simulink library "ebs_rebuild_generic_std"  (R2016a)
settings: Solver=VariableStepAuto  StartTime=0.0  StopTime=10.0  RelTol=1e-3
undefined symbols (not defined in the file): sMP
(part 2 of 2)

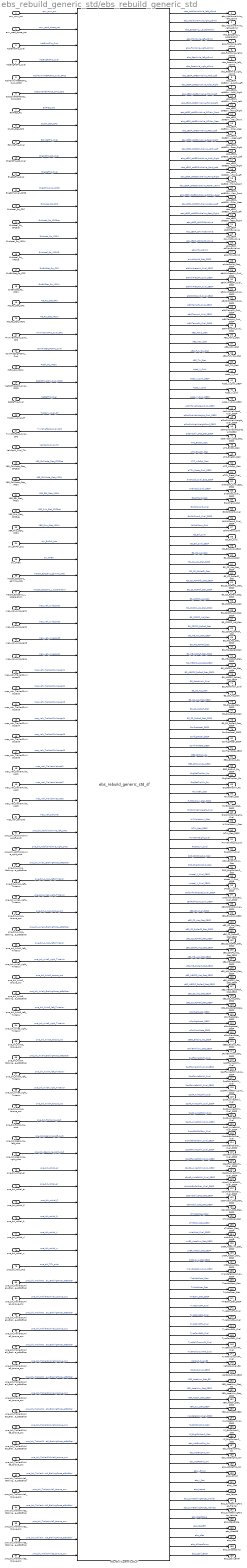
== system ebs_rebuild_generic_std/ebs_rebuild_generic_std ==
  env_curv_pm : Inport
  env_road_slope_pct : Inport  Port=2
  ActlEmotTrq_Cval : Inport  Port=3
  ActlEngPctTrq_Cval : Inport  Port=4
  ActlMaxAvlRetPctTrq_Cval_CPC3 : Inport  Port=5
  aSbspVehBrkForce_Cmd_SDS : Inport  Port=6
  BrkPress_Rq : Inport  Port=7
  Clutch_Stat_CPC : Inport  Port=8
  EdrvRefTrq_Cval : Inport  Port=9
  EngPctTrqActl_Cval : Inport  Port=10
  EngRefTrq_Cval : Inport  Port=11
  EngRPM_Cval_CPC3 : Inport  Port=12
  ExtAccel_Rq_CPC : Inport  Port=13
  ExtAccel_Rq_CPC5ce : Inport  Port=14
  ExtAccel_Rq_VRDU : Inport  Port=15
  ExtAccel_Rq_VRDU3 : Inport  Port=16
  ExtBrkStat_Rq_CPC : Inport  Port=17
  ExtBrkStat_Rq_VRDU : Inport  Port=18
  HB_Rq_Stat_CPC : Inport  Port=19
  HB_Rq_Stat_VRDU : Inport  Port=20
  MinAvlEmotTrq_Cval_CPC : Inport  Port=21
  NomFrictEngPctTrq_Cval : Inport  Port=22
  PkBrk_Rq_VRDU : Inport  Port=23
  RetPctTrqActl2_Cval_CPC3 : Inport  Port=24
  RetRefTrq_Cval : Inport  Port=25
  TrqConv_Cval_PT : Inport  Port=26
  TxInShaftSpd_Cval_CPC : Inport  Port=27
  VehSpd1_Cval_Trlr : Inport  Port=28
  XBR_CtrlMode_Stat_CPC5ce : Inport  Port=29
  XBR_CtrlMode_Stat_VRDU : Inport  Port=30
  XBR_EBI_Stat_VRDU : Inport  Port=31
  XBR_Prio_Stat_CPC5ce : Inport  Port=32
  XBR_Prio_Stat_VRDU : Inport  Port=33
  drv_BrkPdl_pos : Inport  Port=34
  drv_PkBrk : Inport  Port=35
  mec3d_ESCsens_gamma_rate : Inport  Port=36
  mec3d_ESCsens_y_acceleration : Inport  Port=37
  mec_veh_AxleLoad1 : Inport  Port=38
  mec_veh_AxleLoad2 : Inport  Port=39
  mec_veh_AxleLoad3 : Inport  Port=40
  mec_veh_AxleLoad4 : Inport  Port=41
  mec_veh_Trailer02AxleLoad1 : Inport  Port=42
  mec_veh_Trailer02AxleLoad2 : Inport  Port=43
  mec_veh_Trailer02AxleLoad3 : Inport  Port=44
  mec_veh_Trailer02AxleLoad4 : Inport  Port=45
  mec_veh_Trailer02AxleLoad5 : Inport  Port=46
  mec_veh_Trailer02AxleLoad6 : Inport  Port=47
  mec_veh_TrailerAxleLoad1 : Inport  Port=48
  mec_veh_TrailerAxleLoad2 : Inport  Port=49
  mec_veh_TrailerAxleLoad3 : Inport  Port=50
  mec_veh_transVel : Inport  Port=51
  pne_brk_AdditionalAxle_left_pAct : Inport  Port=52
  pne_brk_AdditionalAxle_right_pAct : Inport  Port=53
  pne_brk_Axle1_BrakingForce_at8p5bar : Inport  Port=54
  pne_brk_Axle1_left_Tinterior : Inport  Port=55
  pne_brk_Axle1_right_Tinterior : Inport  Port=56
  pne_brk_Axle1_torque_sns : Inport  Port=57
  pne_brk_Axle2_BrakingForce_at8p5bar : Inport  Port=58
  pne_brk_Axle2_left_Tinterior : Inport  Port=59
  pne_brk_Axle2_right_Tinterior : Inport  Port=60
  pne_brk_Axle2_torque_sns : Inport  Port=61
  pne_brk_Axle3_BrakingForce_at8p5bar : Inport  Port=62
  pne_brk_Axle3_left_Tinterior : Inport  Port=63
  pne_brk_Axle3_right_Tinterior : Inport  Port=64
  pne_brk_Axle3_torque_sns : Inport  Port=65
  pne_brk_Axle4_BrakingForce_at8p5bar : Inport  Port=66
  pne_brk_Axle4_left_Tinterior : Inport  Port=67
  pne_brk_Axle4_right_Tinterior : Inport  Port=68
  pne_brk_Axle4_torque_sns : Inport  Port=69
  pne_brk_FrontAxle_pAct : Inport  Port=70
  pne_brk_RearAxle_left_pAct : Inport  Port=71
  pne_brk_RearAxle_right_pAct : Inport  Port=72
  pne_brk_rotVel_al : Inport  Port=73
  pne_brk_rotVel_ar : Inport  Port=74
  pne_brk_rotVel_fl : Inport  Port=75
  pne_brk_rotVel_fr : Inport  Port=76
  pne_brk_rotVel_rl : Inport  Port=77
  pne_brk_rotVel_rr : Inport  Port=78
  pne_brk_TCV_pAct : Inport  Port=79
  pne_brk_Trailer02Axle1_BrakingForce_at8p5bar : Inport  Port=80
  pne_brk_Trailer02Axle1_torque_sns : Inport  Port=81
  pne_brk_Trailer02Axle2_BrakingForce_at8p5bar : Inport  Port=82
  pne_brk_Trailer02Axle2_torque_sns : Inport  Port=83
  pne_brk_Trailer02Axle3_BrakingForce_at8p5bar : Inport  Port=84
  pne_brk_Trailer02Axle3_torque_sns : Inport  Port=85
  pne_brk_Trailer02Axle4_BrakingForce_at8p5bar : Inport  Port=86
  pne_brk_Trailer02Axle4_torque_sns : Inport  Port=87
  pne_brk_Trailer02Axle5_BrakingForce_at8p5bar : Inport  Port=88
  pne_brk_Trailer02Axle5_torque_sns : Inport  Port=89
  pne_brk_Trailer02Axle6_BrakingForce_at8p5bar : Inport  Port=90
  pne_brk_Trailer02Axle6_torque_sns : Inport  Port=91
  pne_brk_TrailerAxle1_BrakingForce_at8p5bar : Inport  Port=92
  pne_brk_TrailerAxle1_torque_sns : Inport  Port=93
  pne_brk_TrailerAxle2_BrakingForce_at8p5bar : Inport  Port=94
  pne_brk_TrailerAxle2_torque_sns : Inport  Port=95
  pne_brk_TrailerAxle3_BrakingForce_at8p5bar : Inport  Port=96
  pne_brk_TrailerAxle3_torque_sns : Inport  Port=97
  ebs_rebuild_generic_std_sf : S-Function  FunctionName=ebs_rebuild_generic_std_sf  Parameters=s1 s2 p1 p2 p3 p4 p5 p6 p7 p8 p9 p10 p11 p12 p13 p14 p15 p16 p17 p18 p19 p20 p21 p22 p23 p24 p25 p26 p27 p28 p29 p30 p31 p32 p33 p34 p35 p36 p37 p38 p39 p40 p41 p42 p43 p44 p45 p46 p47 p48 p49 p50 p51 p52 p53 p54 p55 p56 p57 p58 p59 p60 p61 p62 p63 p64 p65 p66 p67 p68 p69 p70 p71 p72 p73 p74 p75 p76 p77 p78 p79 p80 p81 p82 p83 p84 p85 p86 p87 p88 p89 p90 p91 p92 p93 p94 p95 p96 p97 p98 p99 p100 p101 p102 p103 p104 p105 p106 p107 p108 p109 p110 p111 p112 p113 p114 p115 p116 p117 p118 p119 p120 p121 p122 p123 p124 p125 p126 p127 p128 p129 p130 p131 p132 p133 p134 p135 p136 p137 p138 p139 p140 p141 p142 p143 p144 p145 p146 p147 p148 p149 p150 p151 p152 p153 p154 p155 p156 p157 p158 p159 p160 p161 p162 p163 p164 p165 p166 p167 p168 p169 p170 p171 p172 p173 p174 p175 p176 p177 p178 p179 p180 p181 p182 p183 p184 p185 p186 p187 p188 p189 p190 p191 p192 p193 p194 p195 p196 p197 p198 p199 p200 p201 p202 p203 p204 p205 p206 p207 p208 p209 p210 p211 p212 p213 p214 p215 p216 p217 p218 p219 p220 p221 p222 p223 p224 p225 p226 p227 p228 p229 p230 p231 p232 p233 p234 p235 p236 p237 p238 p239 p240 p241 p242 p243 p244 p245 p246 p247 p248 p249 p250 p251 p252 p253 p254 p255 p256 p257 p258 p259 p260 p261 p262 p263 p264 p265 p266 p267 p268 p269 p270 p271 p272 p273 p274 p275 p276 p277 p278 p279 p280 p281 p282 p283 p284 p285 p286 p287 p288 p289 p290 p291 p292 p293 p294 p295 p296 p297 p298 p299 p300 p301 p302 p303 p304 p305 p306 p307 p308 p309 p310 p311  SFunctionModules=<binary blob, 502 chars, not shown>  SFunctionDeploymentMode=off  EnableBusSupport=off  mask{s1=s1, s2=s2, initCmd='Parameters_ebs_rebuild_generic_std_sf', p1=p1, p2=p2, p3=p3, p4=p4, p5=p5, p6=p6, p7=p7, p8=p8, p9=p9, p10=p10, p11=p11, p12=p12, p13=p13, p14=p14, p15=p15, p16=p16, p17=p17, p18=p18, p19=p19, p20=p20, p21=p21, p22=p22, p23=p23, p24=p24, p25=p25, p26=p26, p27=p27, p28=p28, p29=p29, p30=p30, p31=p31, p32=p32, p33=p33, p34=p34, p35=p35, p36=p36, p37=p37, p38=p38, p39=p39, p40=p40, p41=p41, p42=p42, p43=p43, p44=p44, p45=p45, p46=p46, p47=p47, p48=p48, p49=p49, p50=p50, p51=p51, p52=p52, p53=p53, p54=p54, p55=p55, p56=p56, p57=p57, p58=p58, p59=p59, p60=p60, p61=p61, p62=p62, p63=p63, p64=p64, p65=p65, p66=p66, p67=p67, p68=p68, p69=p69, p70=p70, p71=p71, p72=p72, p73=p73, p74=p74, p75=p75, p76=p76, p77=p77, p78=p78, p79=p79, p80=p80, p81=p81, p82=p82, p83=p83, p84=p84, p85=p85, p86=p86, p87=p87, p88=p88, p89=p89, p90=p90, p91=p91, p92=p92, p93=p93, p94=p94, p95=p95, p96=p96, p97=p97, p98=p98, p99=p99, p100=p100, p101=p101, p102=p102, p103=p103, p104=p104, p105=p105, p106=p106, p107=p107, p108=p108, p109=p109, p110=p110, p111=p111, p112=p112, p113=p113, p114=p114, p115=p115, p116=p116, p117=p117, p118=p118, p119=p119, p120=p120, p121=p121, p122=p122, p123=p123, p124=p124, p125=p125, p126=p126, p127=p127, p128=p128, p129=p129, p130=p130, p131=p131, p132=p132, p133=p133, p134=p134, p135=p135, p136=p136, p137=p137, p138=p138, p139=p139, p140=p140, p141=p141, p142=p142, p143=p143, p144=p144, p145=p145, p146=p146, p147=p147, p148=p148, p149=p149, p150=p150, p151=p151, p152=p152, p153=p153, p154=p154, p155=p155, p156=p156, p157=p157, p158=p158, p159=p159, p160=p160, p161=p161, p162=p162, p163=p163, p164=p164, p165=p165, p166=p166, p167=p167, p168=p168, p169=p169, p170=p170, p171=p171, p172=p172, p173=p173, p174=p174, p175=p175, p176=p176, p177=p177, p178=p178, p179=p179, p180=p180, p181=p181, p182=p182, p183=p183, p184=p184, p185=p185, p186=p186, p187=p187, p188=p188, p189=p189, p190=p190, p191=p191, p192=p192, p193=p193, p194=p194, p195=p195, p196=p196, p197=p197, p198=p198, p199=p199, p200=p200, p201=p201, p202=p202, p203=p203, p204=p204, p205=p205, p206=p206, p207=p207, p208=p208, p209=p209, p210=p210, p211=p211, p212=p212, p213=p213, p214=p214, p215=p215, p216=p216, p217=p217, p218=p218, p219=p219, p220=p220, p221=p221, p222=p222, p223=p223, p224=p224, p225=p225, p226=p226, p227=p227, p228=p228, p229=p229, p230=p230, p231=p231, p232=p232, p233=p233, p234=p234, p235=p235, p236=p236, p237=p237, p238=p238, p239=p239, p240=p240, p241=p241, p242=p242, p243=p243, p244=p244, p245=p245, p246=p246, p247=p247, p248=p248, p249=p249, p250=p250, p251=p251, p252=p252, p253=p253, p254=p254, p255=p255, p256=p256, p257=p257, p258=p258, p259=p259, p260=p260, p261=p261, p262=p262, p263=p263, p264=p264, p265=p265, p266=p266, p267=p267, p268=p268, p269=p269, p270=p270, p271=p271, p272=p272, p273=p273, p274=p274, p275=p275, p276=p276, p277=p277, p278=p278, p279=p279, p280=p280, p281=p281, p282=p282, p283=p283, p284=p284, p285=p285, p286=p286, p287=p287, p288=p288, p289=p289, p290=p290, p291=p291, p292=p292, p293=p293, p294=p294, p295=p295, p296=p296, p297=p297, p298=p298, p299=p299, p300=p300, p301=p301, p302=p302, p303=p303, p304=p304, p305=p305, p306=p306, p307=p307, p308=p308, p309=p309, p310=p310, p311=p311}
      mask prompts: s1 "Solver Type: settings_iMode [-]"; s2 "Solver Step Size: settings_dt [s]"; initCmd "Initialization command"; p1 "Dimension x-Axis zSoll-Curve [max. 40] export=true name=dim_xAxis_zSoll prio=1 dataSetName=ebs_dummy dataClassType=main dataClassName=main  unit='-' description='Dimension x-Axis zSoll-Curve': BWG.dim_xAxis_zSoll [-]"; p2 "Velocity Offset L1o (km/h) export=true name=ABS_L1o prio=1 dataSetName=veh_dummy dataClassType=veh dataClassName=veh unit='km/h' description='Velocity Offset L1o (km/h)': eBS_veh_Param.ABS_L1o [-]"; p3 "Speed Fraction for Threshold Speed 1 (0.01%) export=true name=ABS_L1v prio=1 dataSetName=veh_dummy dataClassType=veh dataClassName=veh unit='' description='Speed Fraction for Threshold Speed 1 (0.01%)': eBS_veh_Param.ABS_L1v [-]"; p4 "Velocity Offset L2o (km/h) export=true name=ABS_L2o prio=1 dataSetName=veh_dummy dataClassType=veh dataClassName=veh unit='km/h' description='Velocity Offset L2o (km/h)': eBS_veh_Param.ABS_L2o [-]"; p5 "Speed Fraction for Threshold Speed 2 (0.01%) export=true name=ABS_L2v prio=1 dataSetName=veh_dummy dataClassType=veh dataClassName=veh unit='' description='Speed Fraction for Threshold Speed 2 (0.01%)': eBS_veh_Param.ABS_L2v [-]"; p6 "Decceleration Threshold in [g] export=true name=ABS_MinusB prio=1 dataSetName=veh_dummy dataClassType=veh dataClassName=veh unit='' description='Decceleration Threshold in [g]': eBS_veh_Param.ABS_MinusB [-]"; p7 "Acceleration Threshold in [g] export=true name=ABS_PlusB prio=1 dataSetName=veh_dummy dataClassType=veh dataClassName=veh unit='' description='Decceleration Threshold in [g]': eBS_veh_Param.ABS_PlusB [-]"; p8 "Upper Acceleration Threshold in [g] export=true name=ABS_PlusOB prio=1 dataSetName=veh_dummy dataClassType=veh dataClassName=veh unit='' description='Upper Acceleration Threshold in [g]': eBS_veh_Param.ABS_PlusOB [-]"; p9 "Holding Time [ms] export=true name=ABS_THe prio=1 dataSetName=veh_dummy dataClassType=veh dataClassName=veh unit='ms' description='Holding Time [ms]': eBS_veh_Param.ABS_THe [-]"; p10 "Holding Time for Pulsating Pressure Build-Up [ms] export=true name=ABS_TPulHold prio=1 dataSetName=veh_dummy dataClassType=veh dataClassName=veh unit='ms' description='Holding Time for Pulsating Pressure Build-Up [ms]': eBS_veh_Param.ABS_TPulHold [-]"; p11 "Opening Time for Pulsating Pressure Build-Up [ms] export=true name=ABS_TPulOpen prio=1 dataSetName=veh_dummy dataClassType=veh dataClassName=veh unit='ms' description='Opening Time for Pulsating Pressure Build-Up [ms]': eBS_veh_Param.ABS_TPulOpen [-]"; p12 "Minimum Velocity for ABS Activity [km/h] export=true name=ABS_vMin_kmh prio=1 dataSetName=veh_dummy dataClassType=veh dataClassName=veh unit='km/h' description='Minimum Velocity for ABS Activity [km/h]': eBS_veh_Param.ABS_vMin_kmh [-]"; p13 "Trailer ABS Config (0 - none, 1- ABS, 2 - EBS (incl. ABS)), used in pneAux export=true name=flagTrailerABS prio=1 dataSetName=veh_dummy dataClassType=veh dataClassName=veh unit='-' description='Trailer ABS Config (0 - none, 1- ABS, 2 - EBS (incl. ABS))': eBS_veh_Param.flagTrailerABS [-]"; p14 "Dyn. Wheel Radius Front Axle [mm] export=true name=rdynFA prio=1 dataSetName=veh_dummy dataClassType=veh dataClassName=veh unit='mm' description='Dyn. Wheel Radius Front Axle [mm]': eBS_veh_Param.rdynFA [-]"; p15 "Dyn. Wheel Radius Rear Axle [mm] export=true name=rdynRA prio=1 dataSetName=veh_dummy dataClassType=veh dataClassName=veh unit='mm' description='Dyn. Wheel Radius Rear Axle [mm]': eBS_veh_Param.rdynRA [-]"; p16 "Dyn. Wheel Radius Trailer Axle [mm] export=true name=rdynTA prio=1 dataSetName=veh_dummy dataClassType=veh dataClassName=veh unit='mm' description='Dyn. Wheel Radius Trailer Axle [mm]': eBS_veh_Param.rdynTA [-]"; p17 "step Size [s] export=true name=stepSize prio=1 dataSetName=veh_dummy dataClassType=veh dataClassName=veh unit='s' description=' step size [s]': eBS_veh_Param.stepSize [s]"; p18 "ALB Linear Pressure Range p2/p1->1:1 export=true name=ALB_dpMin_bar prio=1 dataSetName=ebs_dummy dataClassType=main dataClassName=main unit=bar description='ALB Linear Pressure Range p2/p1->1:1': eBSParam.ALB_dpMin_bar [-]"; p19 "ALB Maximal Rear Axle Load for p2Max [kg] export=true name=ALB_mRA_Max_kg prio=1 dataSetName=ebs_dummy dataClassType=main dataClassName=main unit=kg description='ALB Maximal Rear Axle Load for p2Max [kg]': eBSParam.ALB_mRA_Max_kg [-]"; p20 "ALB Minimal Rear Axle Load for p2Min [kg] export=true name=ALB_mRA_Min_kg prio=1 dataSetName=ebs_dummy dataClassType=main dataClassName=main unit=kg description='ALB Minimal Rear Axle Load for p2Min [kg]': eBSParam.ALB_mRA_Min_kg [-]"; p21 "ALB Reference Inlet Pressure p1 [bar] export=true name=ALB_p1Ref_bar prio=1 dataSetName=ebs_dummy dataClassType=main dataClassName=main unit=bar description='ALB Reference Inlet Pressure p1 [bar]': eBSParam.ALB_p1Ref_bar [-]"; p22 "ALB Maximum Pressure at mRA_Max_kg [bar] export=true name=ALB_p2Max_bar prio=1 dataSetName=ebs_dummy dataClassType=main dataClassName=main unit=bar description='ALB Maximum Pressure at mRA_Max_kg [bar]': eBSParam.ALB_p2Max_bar [-]"; p23 "ALB Minimum Pressure at mRA_Min [bar] export=true name=ALB_p2Min_bar prio=1 dataSetName=ebs_dummy dataClassType=main dataClassName=main unit=bar description='ALB Minimum Pressure at mRA_Min [bar]': eBSParam.ALB_p2Min_bar [-]"; p24 "Maximum Friction Coefficient Rear Axle export=true name=EBI_mueMax prio=1 dataSetName=ebs_dummy dataClassType=main dataClassName=main unit='-' description='Maximum Friction Coefficient Rear Axle': eBSParam.EBI_mueMax [-]"; p25 "Minum Initial Velocity [km/h] (eBIActive>EBI_vMin_kmh) export=true name=EBI_vMin_kmh prio=1 dataSetName=ebs_dummy dataClassType=main dataClassName=main unit='km/h' description='Minum Initial Velocity [km/h] (eBIActive>EBI_vMin_kmh)': eBSParam.EBI_vMin_kmh [-]"; p26 "Vehicle with ABS-Brake System [0-false,1-true] export=true name=flag_ABS prio=1 dataSetName=ebs_dummy dataClassType=main dataClassName=main unit='-' description='Vehicle with ABS-Brake System [0-false,1-true]': eBSParam.flag_ABS [-]"; p27 "Flag Downhill Drive Test [0-false,1-true] export=true name=flag_DownhillDriveTest prio=1 dataSetName=ebs_dummy dataClassType=main dataClassName=main unit='-' description='Flag Downhill Drive Test [0-false,1-true]': eBSParam.flag_DownhillDriveTest [-]"; p28 "Endurance Brake Integration (EBI) [0-no EBI,1-EBI, base deceleration of 2% by service brake, 2- EBI 100%, 3 - prior endurance brake activation, 4 - EBI Bus mode] export=true name=flag_EBI prio=1 dataSetName=ebs_dummy dataClassType=main dataClassName=main unit='-' description='Endurance Brake Integration (EBI) [0-no EBI,1-EBI, base deceleration of 2% by service brake, 2- EBI 100%, 3 - prior endurance brake activation, 4 - EBI Bus mode]': eBSParam.flag_EBI [-]"; p29 "Slope Compensation Active [0 - false,1 - true] export=true name=flag_SlopeCompActive prio=1 dataSetName=ebs_dummy dataClassType=main dataClassName=main unit='-' description='Slope Compensation Active [0 - false,1 - true]': eBSParam.flag_SlopeCompActive [-]"; p30 "Transmission Ratio EMot - Axle [-] export=true name=mec_iDiffAxle prio=1 dataSetName=ebs_dummy dataClassType=main dataClassName=main unit='' description='Transmission Ratio EMot - Axle [-]': eBSParam.mec_iDiffAxle [-]"; p31 "Recuperation value for full brake pedal actuation [Nm] export=true name=Recuperation_end prio=1 dataSetName=ebs_dummy dataClassType=main dataClassName=main unit=kg description='Recuperation value for inital brake pedal actuation [Nm] ': eBSParam.Recuperation_end [-]"; p32 "Recuperation value for inital brake pedal actuation [Nm] export=true name=Recuperation_initial prio=1 dataSetName=ebs_dummy dataClassType=main dataClassName=main unit=kg description='Recuperation value for inital brake pedal actuation [Nm] ': eBSParam.Recuperation_initial [-]"; p33 "aAutoOpMd_Stat_SBSP export=true name=aAutoOpMd_Stat_SBSP prio=1 dataSetName=std dataClassType=initIO dataClassName=initIO unit='-' description='aAutoOpMd_Stat_SBSP': IO_EBS_InputSignals.aAutoOpMd_Stat_SBSP_0 [-]"; p34 "aBrkAirPressAA_Cval_SBSP export=true name=aBrkAirPressAA_Cval_SBSP prio=1 dataSetName=std dataClassType=initIO dataClassName=initIO unit='kPa' description='aBrkAirPressAA_Cval_SBSP': IO_EBS_InputSignals.aBrkAirPressAA_Cval_SBSP_0 [-]"; p35 "aBrkAirPressFA_Cval_SBSP export=true name=aBrkAirPressFA_Cval_SBSP prio=1 dataSetName=std dataClassType=initIO dataClassName=initIO unit='kPa' description='aBrkAirPressFA_Cval_SBSP': IO_EBS_InputSignals.aBrkAirPressFA_Cval_SBSP_0 [-]"; p36 "aBrkAirPressRA_Cval_SBSP export=true name=aBrkAirPressRA_Cval_SBSP prio=1 dataSetName=std dataClassType=initIO dataClassName=initIO unit='kPa' description='aBrkAirPressRA_Cval_SBSP': IO_EBS_InputSignals.aBrkAirPressRA_Cval_SBSP_0 [-]"; p37 "aBrkPdlPosn3_Cval_SBSP export=true name=aBrkPdlPosn3_Cval_SBSP prio=1 dataSetName=std dataClassType=initIO dataClassName=initIO unit='%' description='aBrkPdlPosn3_Cval_SBSP': IO_EBS_InputSignals.aBrkPdlPosn3_Cval_SBSP_0 [-]"; p38 "aBrkTempFA_Cval_SBSP export=true name=aBrkTempFA_Cval_SBSP prio=1 dataSetName=std dataClassType=initIO dataClassName=initIO unit='degC' description='aBrkTempFA_Cval_SBSP': IO_EBS_InputSignals.aBrkTempFA_Cval_SBSP_0 [-]"; p39 "aBrkTempIA_Cval_SBSP export=true name=aBrkTempIA_Cval_SBSP prio=1 dataSetName=std dataClassType=initIO dataClassName=initIO unit='degC' description='aBrkTempIA_Cval_SBSP': IO_EBS_InputSignals.aBrkTempIA_Cval_SBSP_0 [-]"; p40 "aBrkTempRA_Cval_SBSP export=true name=aBrkTempRA_Cval_SBSP prio=1 dataSetName=std dataClassType=initIO dataClassName=initIO unit='degC' description='aBrkTempRA_Cval_SBSP': IO_EBS_InputSignals.aBrkTempRA_Cval_SBSP_0 [-]"; p41 "ABS_Actv2_Stat export=true name=ABS_Actv2_Stat prio=1 dataSetName=std dataClassType=initIO dataClassName=initIO unit='-' description='ABS_Actv2_Stat': IO_EBS_InputSignals.ABS_Actv2_Stat_0 [-]"; p42 "ABS_Actv_Stat export=true name=ABS_Actv_Stat prio=1 dataSetName=std dataClassType=initIO dataClassName=initIO unit='-' description='ABS_Actv_Stat': IO_EBS_InputSignals.ABS_Actv_Stat_0 [-]"; p43 "ABS_FullyOp_Stat export=true name=ABS_FullyOp_Stat prio=1 dataSetName=std dataClassType=initIO dataClassName=initIO unit='-' description='ABS_FullyOp_Stat': IO_EBS_InputSignals.ABS_FullyOp_Stat_0 [-]"; p44 "ABS_Trlr_Stat export=true name=ABS_Trlr_Stat prio=1 dataSetName=std dataClassType=initIO dataClassName=initIO unit='-' description='ABS_Trlr_Stat': IO_EBS_InputSignals.ABS_Trlr_Stat_0 [-]"; p45 "ABS61449S_E_LongitudAcc, 255 SNA; export=true name=Accel_X_Cval prio=1 dataSetName=std dataClassType=initIO dataClassName=initIO unit='m/s^2' description='ABS61449S_E_LongitudAcc, 255 SNA;': IO_EBS_InputSignals.Accel_X_Cval_0 [-]"; p46 "ABS61449S_E_LongitudAcc, 255 SNA; export=true name=Accel_X_Cval_SBSP prio=1 dataSetName=std dataClassType=initIO dataClassName=initIO unit='m/s^2' description='ABS61449S_E_LongitudAcc, 255 SNA;': IO_EBS_InputSignals.Accel_X_Cval_SBSP_0 [-]"; p47 "Accel_Y_Cval export=true name=Accel_Y_Cval prio=1 dataSetName=std dataClassType=initIO dataClassName=initIO unit=m/s^2 description='Accel_Y_Cval': IO_EBS_InputSignals.Accel_Y_Cval_0 [-]"; p48 "Accel_Y_Cval_SBSP export=true name=Accel_Y_Cval_SBSP prio=1 dataSetName=std dataClassType=initIO dataClassName=initIO unit=m/s^2 description='Accel_Y_Cval_SBSP': IO_EBS_InputSignals.Accel_Y_Cval_SBSP_0 [-]"; p49 "ActlEmotTrq_Cval (init) export=true name=ActlEmotTrq_Cval prio=1 dataSetName=std dataClassType=initIO dataClassName=initIO unit='-' description='ActlEmotTrq_Cval (init)': IO_EBS_InputSignals.ActlEmotTrq_Cval_0 [-]"; p50 "ActlEngPctTrq_Cval export=true name=ActlEngPctTrq_Cval prio=1 dataSetName=std dataClassType=initIO dataClassName=initIO unit='-' description='ActlEngPctTrq_Cval': IO_EBS_InputSignals.ActlEngPctTrq_Cval_0 [-]"; p51 "ActlMaxAvlRetPctTrq_Cval_CPC3 export=true name=ActlMaxAvlRetPctTrq_Cval_CPC3 prio=1 dataSetName=std dataClassType=initIO dataClassName=initIO unit='-' description='ActlMaxAvlRetPctTrq_Cval_CPC3': IO_EBS_InputSignals.ActlMaxAvlRetPctTrq_Cval_CPC3_0 [-]"; p52 "AddInfoVehSped_Cval_SBSP (init) export=true name=AddInfoVehSped_Cval_SBSP prio=1 dataSetName=std dataClassType=initIO dataClassName=initIO unit='' description='AddInfoVehSped_Cval_SBSP': IO_EBS_InputSignals.AddInfoVehSped_Cval_SBSP_0 [-]"; p53 "aGroCmbVehWeight_Cval_SBSP export=true name=aGroCmbVehWeight_Cval_SBSP prio=1 dataSetName=std dataClassType=initIO dataClassName=initIO unit='kg' description='aGroCmbVehWeight_Cval_SBSP': IO_EBS_InputSignals.aGroCmbVehWeight_Cval_SBSP_0 [-]"; p54 "aGroCmbVehWeightConf_SBSP export=true name=aGroCmbVehWeightConf_SBSP prio=1 dataSetName=std dataClassType=initIO dataClassName=initIO unit='%' description='Vehicle Mass estimate confidence factor': IO_EBS_InputSignals.aGroCmbVehWeightConf_SBSP_0 [-]"; p55 "aSbspVehBrkForce_Cmd_SDS export=true name=aSbspVehBrkForce_Cmd_SDS prio=1 dataSetName=std dataClassType=initIO dataClassName=initIO unit='N' description='aSbspVehBrkForce_Cmd_SDS': IO_EBS_InputSignals.aSbspVehBrkForce_Cmd_SDS_0 [-]"; p56 "aStandstill_Dtct_Stat_SBSP export=true name=aStandstill_Dtct_Stat_SBSP prio=1 dataSetName=std dataClassType=initIO dataClassName=initIO unit='-' description='Standstill detected Current state': IO_EBS_InputSignals.aStandstill_Dtct_Stat_SBSP_0 [-]"; p57 "ATC_BrkCtrl_Stat export=true name=ATC_BrkCtrl_Stat prio=1 dataSetName=std dataClassType=initIO dataClassName=initIO unit='-' description='ATC_BrkCtrl_Stat': IO_EBS_InputSignals.ATC_BrkCtrl_Stat_0 [-]"; p58 "ATC_EngCtrl_Stat export=true name=ATC_EngCtrl_Stat prio=1 dataSetName=std dataClassType=initIO dataClassName=initIO unit='-' description='ATC_EngCtrl_Stat': IO_EBS_InputSignals.ATC_EngCtrl_Stat_0 [-]"; p59 "ATC_InfoSgl_Stat export=true name=ATC_InfoSgl_Stat prio=1 dataSetName=std dataClassType=initIO dataClassName=initIO unit='-' description='ATC_InfoSgl_Stat': IO_EBS_InputSignals.ATC_InfoSgl_Stat_0 [-]"; p60 "aTCV_Press_Cval_SBSP export=true name=aTCV_Press_Cval_SBSP prio=1 dataSetName=std dataClassType=initIO dataClassName=initIO unit='kPa' description='aTCV_Press_Cval_SBSP': IO_EBS_InputSignals.aTCV_Press_Cval_SBSP_0 [-]"; p61 "aVehSpd_Cval_E2E_SBSP export=true name=aVehSpd_Cval_E2E_SBSP prio=1 dataSetName=std dataClassType=initIO dataClassName=initIO unit='km/h' description='aVehSpd_Cval_E2E_SBSP': IO_EBS_InputSignals.aVehSpd_Cval_E2E_SBSP_0 [-]"; p62 "aVehSpd_Cval_SBSP export=true name=aVehSpd_Cval_SBSP prio=1 dataSetName=std dataClassType=initIO dataClassName=initIO unit='km/h' description='Vehicle Speed Current value': IO_EBS_InputSignals.aVehSpd_Cval_SBSP_0 [-]"; p63 "BlockTend_Stat export=true name=BlockTend_Stat prio=1 dataSetName=std dataClassType=initIO dataClassName=initIO unit='-' description='BlockTend_Stat': IO_EBS_InputSignals.BlockTend_Stat_0 [-]"; p64 "Brake Pedal Position 3 Current value (an CPC3) export=true name=BrkPdlPosn3_Cval prio=1 dataSetName=std dataClassType=initIO dataClassName=initIO unit='%' description='Brake Pedal Position 3 Current value (an CPC3)': IO_EBS_InputSignals.BrkPdlPosn3_Cval_0 [-]"; p65 "Brake Pedal Position 3 Current value (an CPC3) export=true name=BrkPdlPosn3_Cval_SBSP prio=1 dataSetName=std dataClassType=initIO dataClassName=initIO unit='%' description='Brake Pedal Position 3 Current value (an CPC3) SBSP': IO_EBS_InputSignals.BrkPdlPosn3_Cval_SBSP_0 [-]"; p66 "Brake Pedal Position Current value (an CGW) export=true name=BrkPdlPosn_Cval prio=1 dataSetName=std dataClassType=initIO dataClassName=initIO unit='%' description='Brake Pedal Position Current value (an CGW)': IO_EBS_InputSignals.BrkPdlPosn_Cval_0 [-]"; p67 "BrkPress_Rq export=true name=BrkPress_Rq prio=1 dataSetName=std dataClassType=initIO dataClassName=initIO unit='-' description='BrkPress_Rq': IO_EBS_InputSignals.BrkPress_Rq_0 [-]"; p68 "Brake Current value, 254 ERR; 255 SNA; export=true name=BS_Brk_Cval prio=1 dataSetName=std dataClassType=initIO dataClassName=initIO unit='%' description='Brake Current value, 254 ERR; 255 SNA;': IO_EBS_InputSignals.BS_Brk_Cval_0 [-]"; p69 "Brake Current value, 254 ERR; 255 SNA; export=true name=BS_Brk_Cval_SBSP prio=1 dataSetName=std dataClassType=initIO dataClassName=initIO unit='%' description='Brake Current value, 254 ERR; 255 SNA; SBSP': IO_EBS_InputSignals.BS_Brk_Cval_SBSP_0 [-]"; p70 "BS_CS_Acc_Stat export=true name=BS_CS_Acc_Stat prio=1 dataSetName=std dataClassType=initIO dataClassName=initIO unit='-' description='BS_CSCPC_Acc_Stat': IO_EBS_InputSignals.BS_CS_Acc_Stat_0 [-]"; p71 "BS_CS_Acc_Stat_SBSP export=true name=BS_CS_Acc_Stat_SBSP prio=1 dataSetName=std dataClassType=initIO dataClassName=initIO unit='-' description='BS_CSCPC_Acc_Stat': IO_EBS_InputSignals.BS_CS_Acc_Stat_SBSP_0 [-]"; p72 "BS_CS_RqPerf2_Stat export=true name=BS_CS_RqPerf2_Stat prio=1 dataSetName=std dataClassType=initIO dataClassName=initIO unit='-' description='BS_CS_RqPerf2_Stat': IO_EBS_InputSignals.BS_CS_RqPerf2_Stat_0 [-]"; p73 "BS_CS_RqPerf2_Stat_SBSP export=true name=BS_CS_RqPerf2_Stat_SBSP prio=1 dataSetName=std dataClassType=initIO dataClassName=initIO unit='-' description='BS_CS_RqPerf2_Stat_SBSP': IO_EBS_InputSignals.BS_CS_RqPerf2_Stat_SBSP_0 [-]"; p74 "BS_CS_RqPerf_Stat_SBSP export=true name=BS_CS_RqPerf_Stat_SBSP prio=1 dataSetName=std dataClassType=initIO dataClassName=initIO unit='-' description='BS_CS_RqPerf_Stat_SBSP': IO_EBS_InputSignals.BS_CS_RqPerf_Stat_SBSP_0 [-]"; p75 "BS_CSCPC_Acc_Stat export=true name=BS_CSCPC_Acc_Stat prio=1 dataSetName=std dataClassType=initIO dataClassName=initIO unit='-' description='BS_CSCPC_Acc_Stat': IO_EBS_InputSignals.BS_CSCPC_Acc_Stat_0 [-]"; p76 "BS_CSCPC_Acc_Stat_SBSP export=true name=BS_CSCPC_Acc_Stat_SBSP prio=1 dataSetName=std dataClassType=initIO dataClassName=initIO unit='-' description='BS_CSCPC_Acc_Stat_SBSP': IO_EBS_InputSignals.BS_CSCPC_Acc_Stat_SBSP_0 [-]"; p77 "BS_CSCPC_Intf_Stat export=true name=BS_CSCPC_Intf_Stat prio=1 dataSetName=std dataClassType=initIO dataClassName=initIO unit='-' description='BS_CSCPC_Intf_Stat': IO_EBS_InputSignals.BS_CSCPC_Intf_Stat_0 [-]"; p78 "BS_CSCPC_RqPerf_Stat export=true name=BS_CSCPC_RqPerf_Stat prio=1 dataSetName=std dataClassType=initIO dataClassName=initIO unit='-' description='BS_CSCPC_RqPerf_Stat': IO_EBS_InputSignals.BS_CSCPC_RqPerf_Stat_0 [-]"; p79 "BS_HB_Acc_Stat_SBSP export=true name=BS_HB_Acc_Stat_SBSP prio=1 dataSetName=std dataClassType=initIO dataClassName=initIO unit='-' description='BS_HB_Acc_Stat_SBSP': IO_EBS_InputSignals.BS_HB_Acc_Stat_SBSP_0 [-]"; p80 "Brake Current value, 254 ERR; 255 SNA; export=true name=BS_HB_RqPerf_Stat prio=1 dataSetName=std dataClassType=initIO dataClassName=initIO unit='-' description='Brake Current value, 254 ERR; 255 SNA;': IO_EBS_InputSignals.BS_HB_RqPerf_Stat_0 [-]"; p81 "Brake Current value, 254 ERR; 255 SNA; export=true name=BS_HB_RqPerf_Stat_SBSP prio=1 dataSetName=std dataClassType=initIO dataClassName=initIO unit='-' description='Brake Current value, 254 ERR; 255 SNA; SBSP': IO_EBS_InputSignals.BS_HB_RqPerf_Stat_SBSP_0 [-]"; p82 "BS_HBCPC_Acc_Stat_SBSP export=true name=BS_HBCPC_Acc_Stat_SBSP prio=1 dataSetName=std dataClassType=initIO dataClassName=initIO unit='-' description='BS_HBCPC_Acc_Stat_SBSP': IO_EBS_InputSignals.BS_HBCPC_Acc_Stat_SBSP_0 [-]"; p83 "BS_HBCPC_RqPerf_Stat_SBSP export=true name=BS_HBCPC_RqPerf_Stat_SBSP prio=1 dataSetName=std dataClassType=initIO dataClassName=initIO unit='-' description='BS_HBCPC_RqPerf_Stat_SBSP': IO_EBS_InputSignals.BS_HBCPC_RqPerf_Stat_SBSP_0 [-]"; p84 "Road inclination current value (calculated), 254 ERR; 255 SNA; export=true name=BS_RoadIncln_Cval prio=1 dataSetName=std dataClassType=initIO dataClassName=initIO unit='%' description='Road inclination current value (calculated), 254 ERR; 255 SNA;': IO_EBS_InputSignals.BS_RoadIncln_Cval_0 [-]"; p85 "BS_SS_Acc_Stat export=true name=BS_SS_Acc_Stat prio=1 dataSetName=std dataClassType=initIO dataClassName=initIO unit='-' description='BS_CSCPC_Acc_Stat': IO_EBS_InputSignals.BS_SS_Acc_Stat_0 [-]"; p86 "BS_SS_Acc_Stat_SBSP export=true name=BS_SS_Acc_Stat_SBSP prio=1 dataSetName=std dataClassType=initIO dataClassName=initIO unit='-' description='BS_CSCPC_Acc_Stat': IO_EBS_InputSignals.BS_SS_Acc_Stat_SBSP_0 [-]"; p87 "BS_SS_RqPerf_Stat export=true name=BS_SS_RqPerf_Stat prio=1 dataSetName=std dataClassType=initIO dataClassName=initIO unit='-' description='BS_SS_RqPerf_Stat': IO_EBS_InputSignals.BS_SS_RqPerf_Stat_0 [-]"; p88 "BS_SS_RqPerf_Stat_SBSP export=true name=BS_SS_RqPerf_Stat_SBSP prio=1 dataSetName=std dataClassType=initIO dataClassName=initIO unit='-' description='BS_SS_RqPerf_Stat_SBSP': IO_EBS_InputSignals.BS_SS_RqPerf_Stat_SBSP_0 [-]"; p89 "Clutch_Stat_CPC (init) export=true name=Clutch_Stat_CPC prio=1 dataSetName=std dataClassType=initIO dataClassName=initIO unit='-' description='Clutch_Stat_CPC (init)': IO_EBS_InputSignals.Clutch_Stat_CPC_0 [-]"; p90 "ConfLatAccel_SBSP (init) export=true name=ConfLatAccel_SBSP prio=1 dataSetName=std dataClassType=initIO dataClassName=initIO unit='%' description='ConfLatAccel_SBSP': IO_EBS_InputSignals.ConfLatAccel_SBSP_0 [-]"; p91 "ConfLgtAccel_SBSP (init) export=true name=ConfLgtAccel_SBSP prio=1 dataSetName=std dataClassType=initIO dataClassName=initIO unit='%' description='ConfLgtAccel_SBSP': IO_EBS_InputSignals.ConfLgtAccel_SBSP_0 [-]"; p92 "ConfYawRate_SBSP (init) export=true name=ConfYawRate_SBSP prio=1 dataSetName=std dataClassType=initIO dataClassName=initIO unit='%' description='ConfYawRate_SBSP': IO_EBS_InputSignals.ConfYawRate_SBSP_0 [-]"; p93 "drv_BrkPdl_pos export=true name=drv_BrkPdl_pos prio=1 dataSetName=std dataClassType=initIO dataClassName=initIO unit='-' description='drv_BrkPdl_pos': IO_EBS_InputSignals.drv_BrkPdl_pos_0 [-]"; p94 "drv_PkBrk export=true name=drv_PkBrk prio=1 dataSetName=std dataClassType=initIO dataClassName=initIO unit='-' description='drv_PkBrk': IO_EBS_InputSignals.drv_PkBrk_0 [-]"; p95 "ebs_ActlEmotTrq_Nm export=true name=ebs_ActlEmotTrq_Nm prio=1 dataSetName=std dataClassType=initIO dataClassName=initIO unit=Nm description='ebs_ActlEmotTrq_Nm': IO_EBS_InputSignals.ebs_ActlEmotTrq_Nm_0 [-]"; p96 "ebs_ActlEngTrq_Nm export=true name=ebs_ActlEngTrq_Nm prio=1 dataSetName=std dataClassType=initIO dataClassName=initIO unit=Nm description='ebs_ActlEngTrq_Nm': IO_EBS_InputSignals.ebs_ActlEngTrq_Nm_0 [-]"; p97 "ebs_ActlRetTrq_Nm export=true name=ebs_ActlRetTrq_Nm prio=1 dataSetName=std dataClassType=initIO dataClassName=initIO unit=Nm description='ebs_ActlRetTrq_Nm': IO_EBS_InputSignals.ebs_ActlRetTrq_Nm_0 [-]"; p98 "ebs_AdditionalAxle_left_pDmd (init) export=true name=ebs_AdditionalAxle_left_pDmd prio=1 dataSetName=std dataClassType=initIO dataClassName=initIO unit='-' description='ebs_AdditionalAxle_left_pDmd': IO_EBS_InputSignals.ebs_AdditionalAxle_left_pDmd_0 [-]"; p99 "ebs_AdditionalAxle_right_pDmd (init) export=true name=ebs_AdditionalAxle_right_pDmd prio=1 dataSetName=std dataClassType=initIO dataClassName=initIO unit='-' description='ebs_AdditionalAxle_right_pDmd': IO_EBS_InputSignals.ebs_AdditionalAxle_right_pDmd_0 [-]"; p100 "EBS Brake Switch 2 Request state for DTR+, 0 NPSD; 1 PSD; 2 ERR; 3 SNA; export=true name=EBS_BrkSw2_Rq prio=1 dataSetName=std dataClassType=initIO dataClassName=initIO unit='-' description='EBS Brake Switch 2 Request state for DTR+, 0 NPSD; 1 PSD; 2 ERR; 3 SNA;': IO_EBS_InputSignals.EBS_BrkSw2_Rq_0 [-]"; p101 "EBS Brake Switch 2 Request state for DTR+, 0 NPSD; 1 PSD; 2 ERR; 3 SNA; export=true name=EBS_BrkSw2_Rq_SBSP prio=1 dataSetName=std dataClassType=initIO dataClassName=initIO unit='-' description='EBS Brake Switch 2 Request state for DTR+, 0 NPSD; 1 PSD; 2 ERR; 3 SNA;': IO_EBS_InputSignals.EBS_BrkSw2_Rq_SBSP_0 [-]"; p102 "ebs_ESCsens_y_acceleration export=true name=ebs_ESCsens_y_acceleration prio=1 dataSetName=std dataClassType=initIO dataClassName=initIO unit='m/s^2' description='ebs_ESCsens_y_acceleration': IO_EBS_InputSignals.ebs_ESCsens_y_acceleration_0 [-]"; p103 "ebs_FrontAxle_left_pDmd (init) export=true name=ebs_FrontAxle_left_pDmd prio=1 dataSetName=std dataClassType=initIO dataClassName=initIO unit='-' description='ebs_FrontAxle_left_pDmd': IO_EBS_InputSignals.ebs_FrontAxle_left_pDmd_0 [-]"; p104 "ebs_FrontAxle_right_pDmd (init) export=true name=ebs_FrontAxle_right_pDmd prio=1 dataSetName=std dataClassType=initIO dataClassName=initIO unit='-' description='ebs_FrontAxle_right_pDmd': IO_EBS_InputSignals.ebs_FrontAxle_right_pDmd_0 [-]"; p105 "ebs_i_Emot export=true name=ebs_i_Emot prio=1 dataSetName=std dataClassType=initIO dataClassName=initIO unit='-' description='ebs_i_Emot': IO_EBS_InputSignals.ebs_i_Emot_0 [-]"; p106 "ebs_i_Ret export=true name=ebs_i_Ret prio=1 dataSetName=std dataClassType=initIO dataClassName=initIO unit='-' description='ebs_i_Ret': IO_EBS_InputSignals.ebs_i_Ret_0 [-]"; p107 "ebs_kappa export=true name=ebs_kappa prio=1 dataSetName=std dataClassType=initIO dataClassName=initIO unit='-' description='ebs_kappa': IO_EBS_InputSignals.ebs_kappa_0 [-]"; p108 "ebs_RearAxle_left_pDmd (init) export=true name=ebs_RearAxle_left_pDmd prio=1 dataSetName=std dataClassType=initIO dataClassName=initIO unit='-' description='ebs_RearAxle_left_pDmd': IO_EBS_InputSignals.ebs_RearAxle_left_pDmd_0 [-]"; p109 "ebs_RearAxle_right_pDmd (init) export=true name=ebs_RearAxle_right_pDmd prio=1 dataSetName=std dataClassType=initIO dataClassName=initIO unit='-' description='ebs_RearAxle_right_pDmd': IO_EBS_InputSignals.ebs_RearAxle_right_pDmd_0 [-]"; p110 "ebs_sBSP_stABSInValve_Addl_Left export=true name=ebs_sBSP_stABSInValve_Addl_Left prio=1 dataSetName=std dataClassType=initIO dataClassName=initIO unit='-' description='ebs_sBSP_stABSInValve_Addl_Left': IO_EBS_InputSignals.ebs_sBSP_stABSInValve_Addl_Left_0 [-]"; p111 "ebs_sBSP_stABSInValve_Addl_Right export=true name=ebs_sBSP_stABSInValve_Addl_Right prio=1 dataSetName=std dataClassType=initIO dataClassName=initIO unit='-' description='ebs_sBSP_stABSInValve_Addl_Right': IO_EBS_InputSignals.ebs_sBSP_stABSInValve_Addl_Right_0 [-]"; p112 "ebs_sBSP_stABSInValve_Front_Left export=true name=ebs_sBSP_stABSInValve_Front_Left prio=1 dataSetName=std dataClassType=initIO dataClassName=initIO unit='-' description='ebs_sBSP_stABSInValve_Front_Left': IO_EBS_InputSignals.ebs_sBSP_stABSInValve_Front_Left_0 [-]"; p113 "ebs_sBSP_stABSInValve_Front_Right export=true name=ebs_sBSP_stABSInValve_Front_Right prio=1 dataSetName=std dataClassType=initIO dataClassName=initIO unit='-' description='ebs_sBSP_stABSInValve_Front_Right': IO_EBS_InputSignals.ebs_sBSP_stABSInValve_Front_Right_0 [-]"; p114 "ebs_sBSP_stABSInValve_RCMax_Front (init),   export=true name=ebs_sBSP_stABSInValve_RCMax_Front prio=1 dataSetName=std dataClassType=initIO dataClassName=initIO unit='-' description=' ': IO_EBS_InputSignals.ebs_sBSP_stABSInValve_RCMax_Front_0 [-]"; p115 "ebs_sBSP_stABSInValve_RCMax_Rear (init),   export=true name=ebs_sBSP_stABSInValve_RCMax_Rear prio=1 dataSetName=std dataClassType=initIO dataClassName=initIO unit='-' description=' ': IO_EBS_InputSignals.ebs_sBSP_stABSInValve_RCMax_Rear_0 [-]"; p116 "ebs_sBSP_stABSInValve_Rear_Left export=true name=ebs_sBSP_stABSInValve_Rear_Left prio=1 dataSetName=std dataClassType=initIO dataClassName=initIO unit='-' description='ebs_sBSP_stABSInValve_Rear_Left': IO_EBS_InputSignals.ebs_sBSP_stABSInValve_Rear_Left_0 [-]"; p117 "ebs_sBSP_stABSInValve_Rear_Right export=true name=ebs_sBSP_stABSInValve_Rear_Right prio=1 dataSetName=std dataClassType=initIO dataClassName=initIO unit='-' description='ebs_sBSP_stABSInValve_Rear_Right': IO_EBS_InputSignals.ebs_sBSP_stABSInValve_Rear_Right_0 [-]"; p118 "ebs_sBSP_stABSOutValve_Addl_Left export=true name=ebs_sBSP_stABSOutValve_Addl_Left prio=1 dataSetName=std dataClassType=initIO dataClassName=initIO unit='-' description='ebs_sBSP_stABSOutValve_Addl_Left': IO_EBS_InputSignals.ebs_sBSP_stABSOutValve_Addl_Left_0 [-]"; p119 "ebs_sBSP_stABSOutValve_Addl_Right export=true name=ebs_sBSP_stABSOutValve_Addl_Right prio=1 dataSetName=std dataClassType=initIO dataClassName=initIO unit='-' description='ebs_sBSP_stABSOutValve_Addl_Right': IO_EBS_InputSignals.ebs_sBSP_stABSOutValve_Addl_Right_0 [-]"; p120 "ebs_sBSP_stABSOutValve_Front_Left export=true name=ebs_sBSP_stABSOutValve_Front_Left prio=1 dataSetName=std dataClassType=initIO dataClassName=initIO unit='-' description='ebs_sBSP_stABSOutValve_Front_Left': IO_EBS_InputSignals.ebs_sBSP_stABSOutValve_Front_Left_0 [-]"; p121 "ebs_sBSP_stABSOutValve_Front_Right export=true name=ebs_sBSP_stABSOutValve_Front_Right prio=1 dataSetName=std dataClassType=initIO dataClassName=initIO unit='-' description='ebs_sBSP_stABSOutValve_Front_Right': IO_EBS_InputSignals.ebs_sBSP_stABSOutValve_Front_Right_0 [-]"; p122 "ebs_sBSP_stABSOutValve_RCMax_Front (init),   export=true name=ebs_sBSP_stABSOutValve_RCMax_Front prio=1 dataSetName=std dataClassType=initIO dataClassName=initIO unit='-' description=' ': IO_EBS_InputSignals.ebs_sBSP_stABSOutValve_RCMax_Front_0 [-]"; p123 "ebs_sBSP_stABSOutValve_RCMax_Rear (init),   export=true name=ebs_sBSP_stABSOutValve_RCMax_Rear prio=1 dataSetName=std dataClassType=initIO dataClassName=initIO unit='-' description=' ': IO_EBS_InputSignals.ebs_sBSP_stABSOutValve_RCMax_Rear_0 [-]"; p124 "ebs_sBSP_stABSOutValve_Rear_Left export=true name=ebs_sBSP_stABSOutValve_Rear_Left prio=1 dataSetName=std dataClassType=initIO dataClassName=initIO unit='-' description='ebs_sBSP_stABSOutValve_Rear_Left': IO_EBS_InputSignals.ebs_sBSP_stABSOutValve_Rear_Left_0 [-]"; p125 "ebs_sBSP_stABSOutValve_Rear_Right export=true name=ebs_sBSP_stABSOutValve_Rear_Right prio=1 dataSetName=std dataClassType=initIO dataClassName=initIO unit='-' description='ebs_sBSP_stABSOutValve_Rear_Right': IO_EBS_InputSignals.ebs_sBSP_stABSOutValve_Rear_Right_0 [-]"; p126 "ebs_sBSP_stAPCVBuValve export=true name=ebs_sBSP_stAPCVBuValve prio=1 dataSetName=std dataClassType=initIO dataClassName=initIO unit='-' description='ebs_sBSP_stAPCVBuValve': IO_EBS_InputSignals.ebs_sBSP_stAPCVBuValve_0 [-]"; p127 "ebs_sBSP_stAxmoBuValve export=true name=ebs_sBSP_stAxmoBuValve prio=1 dataSetName=std dataClassType=initIO dataClassName=initIO unit='-' description='ebs_sBSP_stAxmoBuValve': IO_EBS_InputSignals.ebs_sBSP_stAxmoBuValve_0 [-]"; p128 "ebs_sBSP_stCMaxBuValve export=true name=ebs_sBSP_stCMaxBuValve prio=1 dataSetName=std dataClassType=initIO dataClassName=initIO unit='-' description='ebs_sBSP_stCMaxBuValve': IO_EBS_InputSignals.ebs_sBSP_stCMaxBuValve_0 [-]"; p129 "ebs_SumBrakingForces_Trailer (init) export=true name=ebs_SumBrakingForces_Trailer prio=1 dataSetName=std dataClassType=initIO dataClassName=initIO unit='-' description='ebs_SumBrakingForces_Trailer': IO_EBS_InputSignals.ebs_SumBrakingForces_Trailer_0 [-]"; p130 "ebs_SumBrakingForces_Vehicle (init) export=true name=ebs_SumBrakingForces_Vehicle prio=1 dataSetName=std dataClassType=initIO dataClassName=initIO unit='-' description='ebs_SumBrakingForces_Vehicle': IO_EBS_InputSignals.ebs_SumBrakingForces_Vehicle_0 [-]"; p131 "ebs_TCV_pDmd (init) export=true name=ebs_TCV_pDmd prio=1 dataSetName=std dataClassType=initIO dataClassName=initIO unit='-' description='ebs_TCV_pDmd': IO_EBS_InputSignals.ebs_TCV_pDmd_0 [-]"; p132 "ebs_zReqBrake export=true name=ebs_zReqBrake prio=1 dataSetName=std dataClassType=initIO dataClassName=initIO unit='-' description='ebs_zReqBrake': IO_EBS_InputSignals.ebs_zReqBrake_0 [-]"; p133 "ebs_zReqEB export=true name=ebs_zReqEB prio=1 dataSetName=std dataClassType=initIO dataClassName=initIO unit='-' description='ebs_zReqEB': IO_EBS_InputSignals.ebs_zReqEB_0 [-]"; p134 "ebs_zRet export=true name=ebs_zRet prio=1 dataSetName=std dataClassType=initIO dataClassName=initIO unit='-' description='ebs_zRet': IO_EBS_InputSignals.ebs_zRet_0 [-]"; p135 "ebs_zSlopeComp export=true name=ebs_zSlopeComp prio=1 dataSetName=std dataClassType=initIO dataClassName=initIO unit='-' description='ebs_zSlopeComp': IO_EBS_InputSignals.ebs_zSlopeComp_0 [-]"; p136 "ebs_zSoll_BWG export=true name=ebs_zSoll_BWG prio=1 dataSetName=std dataClassType=initIO dataClassName=initIO unit='-' description='ebs_zSoll_BWG': IO_EBS_InputSignals.ebs_zSoll_BWG_0 [-]"; p137 "EdrvRefTrq_Cval (init) export=true name=EdrvRefTrq_Cval prio=1 dataSetName=std dataClassType=initIO dataClassName=initIO unit='-' description='EdrvRefTrq_Cval (init)': IO_EBS_InputSignals.EdrvRefTrq_Cval_0 [-]"; p138 "EngPctTrqActl_Cval export=true name=EngPctTrqActl_Cval prio=1 dataSetName=std dataClassType=initIO dataClassName=initIO unit='-' description='EngPctTrqActl_Cval': IO_EBS_InputSignals.EngPctTrqActl_Cval_0 [-]"; p139 "EngRefTrq_Cval export=true name=EngRefTrq_Cval prio=1 dataSetName=std dataClassType=initIO dataClassName=initIO unit='-' description='EngRefTrq_Cval': IO_EBS_InputSignals.EngRefTrq_Cval_0 [-]"; p140 "EngRetTrqMax_Rq (toCAN) export=true name=EngRetTrqMax_Rq prio=1 dataSetName=std dataClassType=initIO dataClassName=initIO unit='-' description='EngRetTrqMax_Rq (toCAN)': IO_EBS_InputSignals.EngRetTrqMax_Rq_0 [-]"; p141 "EngRetTrqMin_Rq (to CAN) export=true name=EngRetTrqMin_Rq prio=1 dataSetName=std dataClassType=initIO dataClassName=initIO unit='-' description='EngRetTrqMin_Rq (to CAN)': IO_EBS_InputSignals.EngRetTrqMin_Rq_0 [-]"; p142 "Engine RPM Current value from CPC export=true name=EngRPM_Cval_CPC3 prio=1 dataSetName=std dataClassType=initIO dataClassName=initIO unit='-' description='Engine RPM Current value from CPC': IO_EBS_InputSignals.EngRPM_Cval_CPC3_0 [-]"; p143 "curvature of road [1/m] export=true name=env_curv_pm prio=1 dataSetName=std dataClassType=initIO dataClassName=initIO unit='-' description='curvature of road [1/m]': IO_EBS_InputSignals.env_curv_pm_0 [-]"; p144 "slope of road [%] export=true name=env_road_slope_pct prio=1 dataSetName=std dataClassType=initIO dataClassName=initIO unit='-' description='slope of road [%]': IO_EBS_InputSignals.env_road_slope_pct_0 [-]"; p145 "ExtAccel_Rq_CPC5ce [m/s^2] export=true name=ExtAccel_Rq_CPC5ce prio=1 dataSetName=std dataClassType=initIO dataClassName=initIO unit='-' description='ExtAccel_Rq_CPC5ce [m/s^2]': IO_EBS_InputSignals.ExtAccel_Rq_CPC5ce_0 [-]"; p146 "ExtAccel_Rq_CPC [m/s^2] export=true name=ExtAccel_Rq_CPC prio=1 dataSetName=std dataClassType=initIO dataClassName=initIO unit='-' description='ExtAccel_Rq_CPC [m/s^2]': IO_EBS_InputSignals.ExtAccel_Rq_CPC_0 [-]"; p147 "ExtAccel_Rq_VRDU3 export=true name=ExtAccel_Rq_VRDU3 prio=1 dataSetName=std dataClassType=initIO dataClassName=initIO unit='m/s^2' description='ACC External Acceleration Demand': IO_EBS_InputSignals.ExtAccel_Rq_VRDU3_0 [-]"; p148 "ExtAccel_Rq_VRDU [m/s^2] export=true name=ExtAccel_Rq_VRDU prio=1 dataSetName=std dataClassType=initIO dataClassName=initIO unit='-' description='ExtAccel_Rq_VRDU [m/s^2]': IO_EBS_InputSignals.ExtAccel_Rq_VRDU_0 [-]"; p149 "ExtBrkStat_Rq_CPC [-] export=true name=ExtBrkStat_Rq_CPC prio=1 dataSetName=std dataClassType=initIO dataClassName=initIO unit='-' description='ExtBrkStat_Rq_CPC [-]': IO_EBS_InputSignals.ExtBrkStat_Rq_CPC_0 [-]"; p150 "ExtBrkStat_Rq_VRDU [-] export=true name=ExtBrkStat_Rq_VRDU prio=1 dataSetName=std dataClassType=initIO dataClassName=initIO unit='-' description='ExtBrkStat_Rq_VRDU [-]': IO_EBS_InputSignals.ExtBrkStat_Rq_VRDU_0 [-]"; p151 "FoundBrk_Stat service brake is:   0 --> inaktive , 1 --> aktive, 4 --> sna export=true name=FoundBrk_Stat prio=1 dataSetName=std dataClassType=initIO dataClassName=initIO unit='-' description='FoundBrk_Stat, service brake is:   0 --> inaktive , 1 --> aktive, 4 --> sna': IO_EBS_InputSignals.FoundBrk_Stat_0 [-]"; p152 "FullBrkAllow_Stat_SBSP export=true name=FullBrkAllow_Stat_SBSP prio=1 dataSetName=std dataClassType=initIO dataClassName=initIO unit='-' description='FullBrkAllow_Stat_SBSP': IO_EBS_InputSignals.FullBrkAllow_Stat_SBSP_0 [-]"; p153 "GroCmbVehWeight_Cval (init) export=true name=GroCmbVehWeight_Cval prio=1 dataSetName=std dataClassType=initIO dataClassName=initIO unit=kg description='GroCmbVehWeight_Cval': IO_EBS_InputSignals.GroCmbVehWeight_Cval_0 [-]"; p154 "HB_Rq_Stat_CPC export=true name=HB_Rq_Stat_CPC prio=1 dataSetName=std dataClassType=initIO dataClassName=initIO unit='-' description='HB_Rq_Stat_CPC': IO_EBS_InputSignals.HB_Rq_Stat_CPC_0 [-]"; p155 "HB_Rq_Stat_VRDU export=true name=HB_Rq_Stat_VRDU prio=1 dataSetName=std dataClassType=initIO dataClassName=initIO unit='-' description='HB_Rq_Stat_VRDU': IO_EBS_InputSignals.HB_Rq_Stat_VRDU_0 [-]"; p156 "Hill Holder Availability Current State, 0 HH_AVL; 1 HH_ACTV_NOT_FF; 2 HH_MF; 3 SNA; export=true name=HillHolderAvl_Stat prio=1 dataSetName=std dataClassType=initIO dataClassName=initIO unit='-' description='Hill Holder Availability Current State, 0 HH_AVL; 1 HH_ACTV_NOT_FF; 2 HH_MF; 3 SNA;': IO_EBS_InputSignals.HillHolderAvl_Stat_0 [-]"; p157 "mec3d_ESCsens_gamma_rate export=true name=mec3d_ESCsens_gamma_rate prio=1 dataSetName=std dataClassType=initIO dataClassName=initIO unit='rad/s' description='mec3d_ESCsens_gamma_rate': IO_EBS_InputSignals.mec3d_ESCsens_gamma_rate_0 [-]"; p158 "mec3d_ESCsens_y_acceleration export=true name=mec3d_ESCsens_y_acceleration prio=1 dataSetName=std dataClassType=initIO dataClassName=initIO unit='m/s^2' description='mec3d_ESCsens_y_acceleration': IO_EBS_InputSignals.mec3d_ESCsens_y_acceleration_0 [-]"; p159 "mec_veh_AxleLoad1 (init) export=true name=mec_veh_AxleLoad1 prio=1 dataSetName=std dataClassType=initIO dataClassName=initIO unit=kg description='mec_veh_AxleLoad1': IO_EBS_InputSignals.mec_veh_AxleLoad1_0 [-]"; p160 "mec_veh_AxleLoad2 (init) export=true name=mec_veh_AxleLoad2 prio=1 dataSetName=std dataClassType=initIO dataClassName=initIO unit=kg description='mec_veh_AxleLoad2': IO_EBS_InputSignals.mec_veh_AxleLoad2_0 [-]"; p161 "mec_veh_AxleLoad3 (init) export=true name=mec_veh_AxleLoad3 prio=1 dataSetName=std dataClassType=initIO dataClassName=initIO unit=kg description='mec_veh_AxleLoad3': IO_EBS_InputSignals.mec_veh_AxleLoad3_0 [-]"; p162 "mec_veh_AxleLoad4 (init) export=true name=mec_veh_AxleLoad4 prio=1 dataSetName=std dataClassType=initIO dataClassName=initIO unit=kg description='mec_veh_AxleLoad4': IO_EBS_InputSignals.mec_veh_AxleLoad4_0 [-]"; p163 "mec_veh_Trailer02AxleLoad1 (init) export=true name=mec_veh_Trailer02AxleLoad1 prio=1 dataSetName=std dataClassType=initIO dataClassName=initIO unit=kg description='mec_veh_Trailer02AxleLoad1': IO_EBS_InputSignals.mec_veh_Trailer02AxleLoad1_0 [-]"; p164 "mec_veh_Trailer02AxleLoad2 (init) export=true name=mec_veh_Trailer02AxleLoad2 prio=1 dataSetName=std dataClassType=initIO dataClassName=initIO unit=kg description='mec_veh_Trailer02AxleLoad2': IO_EBS_InputSignals.mec_veh_Trailer02AxleLoad2_0 [-]"; p165 "mec_veh_Trailer02AxleLoad3 (init) export=true name=mec_veh_Trailer02AxleLoad3 prio=1 dataSetName=std dataClassType=initIO dataClassName=initIO unit=kg description='mec_veh_Trailer02AxleLoad3': IO_EBS_InputSignals.mec_veh_Trailer02AxleLoad3_0 [-]"; p166 "mec_veh_Trailer02AxleLoad4 (init) export=true name=mec_veh_Trailer02AxleLoad4 prio=1 dataSetName=std dataClassType=initIO dataClassName=initIO unit=kg description='mec_veh_Trailer02AxleLoad4': IO_EBS_InputSignals.mec_veh_Trailer02AxleLoad4_0 [-]"; p167 "mec_veh_Trailer02AxleLoad5 (init) export=true name=mec_veh_Trailer02AxleLoad5 prio=1 dataSetName=std dataClassType=initIO dataClassName=initIO unit=kg description='mec_veh_Trailer02AxleLoad5': IO_EBS_InputSignals.mec_veh_Trailer02AxleLoad5_0 [-]"; p168 "mec_veh_Trailer02AxleLoad6 (init) export=true name=mec_veh_Trailer02AxleLoad6 prio=1 dataSetName=std dataClassType=initIO dataClassName=initIO unit=kg description='mec_veh_Trailer02AxleLoad6': IO_EBS_InputSignals.mec_veh_Trailer02AxleLoad6_0 [-]"; p169 "mec_veh_TrailerAxleLoad1 (init) export=true name=mec_veh_TrailerAxleLoad1 prio=1 dataSetName=std dataClassType=initIO dataClassName=initIO unit=kg description='mec_veh_TrailerAxleLoad1': IO_EBS_InputSignals.mec_veh_TrailerAxleLoad1_0 [-]"; p170 "mec_veh_TrailerAxleLoad2 (init) export=true name=mec_veh_TrailerAxleLoad2 prio=1 dataSetName=std dataClassType=initIO dataClassName=initIO unit=kg description='mec_veh_TrailerAxleLoad2': IO_EBS_InputSignals.mec_veh_TrailerAxleLoad2_0 [-]"; p171 "mec_veh_TrailerAxleLoad3 (init) export=true name=mec_veh_TrailerAxleLoad3 prio=1 dataSetName=std dataClassType=initIO dataClassName=initIO unit=kg description='mec_veh_TrailerAxleLoad3': IO_EBS_InputSignals.mec_veh_TrailerAxleLoad3_0 [-]"; p172 "mec_veh_transVel export=true name=mec_veh_transVel prio=1 dataSetName=std dataClassType=initIO dataClassName=initIO unit='-' description='mec_veh_transVel': IO_EBS_InputSignals.mec_veh_transVel_0 [-]"; p173 "MinAvlEmotTrq_Cval_CPC (init) export=true name=MinAvlEmotTrq_Cval_CPC prio=1 dataSetName=std dataClassType=initIO dataClassName=initIO unit='-' description='MinAvlEmotTrq_Cval_CPC (init)': IO_EBS_InputSignals.MinAvlEmotTrq_Cval_CPC_0 [-]"; p174 "NomFrictEngPctTrq_Cval export=true name=NomFrictEngPctTrq_Cval prio=1 dataSetName=std dataClassType=initIO dataClassName=initIO unit='-' description='NomFrictEngPctTrq_Cval': IO_EBS_InputSignals.NomFrictEngPctTrq_Cval_0 [-]"; p175 "NrTrlr_Stat_SBSP (init) export=true name=NrTrlr_Stat_SBSP prio=1 dataSetName=std dataClassType=initIO dataClassName=initIO unit='' description='NrTrlr_Stat_SBSP': IO_EBS_InputSignals.NrTrlr_Stat_SBSP_0 [-]"; p176 "PkBrk_Rq_VRDU export=true name=PkBrk_Rq_VRDU prio=1 dataSetName=std dataClassType=initIO dataClassName=initIO unit='-' description='PkBrk_Rq_VRDU': IO_EBS_InputSignals.PkBrk_Rq_VRDU_0 [-]"; p177 "Front axle: acting pressure export=true name=pne_brk_AdditionalAxle_left_pAct prio=1 dataSetName=std dataClassType=initIO dataClassName=initIO unit='bar' description='actual pressure Additional leftt at 2k-AXMO': IO_EBS_InputSignals.pne_brk_AdditionalAxle_left_pAct_0 [-]"; p178 "Front axle: acting pressure export=true name=pne_brk_AdditionalAxle_right_pAct prio=1 dataSetName=std dataClassType=initIO dataClassName=initIO unit='bar' description='actual pressure Additional right at 2k-AXMO': IO_EBS_InputSignals.pne_brk_AdditionalAxle_right_pAct_0 [-]"; p179 "pne_brk_Axle1_BrakingForce_at8p5bar [N] (init) export=true name=pne_brk_Axle1_BrakingForce_at8p5bar prio=1 dataSetName=std dataClassType=initIO dataClassName=initIO unit=N description='pne_brk_Axle1_BrakingForce_at8p5bar [N] (init)': IO_EBS_InputSignals.pne_brk_Axle1_BrakingForce_at8p5bar_0 [-]"; p180 "axle 1 left temperature of the friction area [degC] (init) export=true name=pne_brk_Axle1_left_Tinterior prio=1 dataSetName=std dataClassType=initIO dataClassName=initIO unit=degC description='axle 1 left inner temperature [degC] (init)': IO_EBS_InputSignals.pne_brk_Axle1_left_Tinterior_0 [-]"; p181 "axle 1 right temperature of the friction area [degC] (init) export=true name=pne_brk_Axle1_right_Tinterior prio=1 dataSetName=std dataClassType=initIO dataClassName=initIO unit=degC description='axle 1 right inner temperature [degC] (init)': IO_EBS_InputSignals.pne_brk_Axle1_right_Tinterior_0 [-]"; p182 "pne_brk_Axle1_torque_sns export=true name=pne_brk_Axle1_torque_sns prio=1 dataSetName=std dataClassType=initIO dataClassName=initIO unit='-' description='pne_brk_Axle1_torque_sns': IO_EBS_InputSignals.pne_brk_Axle1_torque_sns_0 [-]"; p183 "pne_brk_Axle2_BrakingForce_at8p5bar [N] (init) export=true name=pne_brk_Axle2_BrakingForce_at8p5bar prio=1 dataSetName=std dataClassType=initIO dataClassName=initIO unit=N description='pne_brk_Axle2_BrakingForce_at8p5bar [N] (init)': IO_EBS_InputSignals.pne_brk_Axle2_BrakingForce_at8p5bar_0 [-]"; p184 "axle 2 left temperature of the friction area [degC] (init) export=true name=pne_brk_Axle2_left_Tinterior prio=1 dataSetName=std dataClassType=initIO dataClassName=initIO unit=degC description='axle 1 left inner temperature [degC] (init)': IO_EBS_InputSignals.pne_brk_Axle2_left_Tinterior_0 [-]"; p185 "axle 2 right temperature of the friction area [degC] (init) export=true name=pne_brk_Axle2_right_Tinterior prio=1 dataSetName=std dataClassType=initIO dataClassName=initIO unit=degC description='axle 1 right inner temperature [degC] (init)': IO_EBS_InputSignals.pne_brk_Axle2_right_Tinterior_0 [-]"; p186 "pne_brk_Axle2_torque_sns export=true name=pne_brk_Axle2_torque_sns prio=1 dataSetName=std dataClassType=initIO dataClassName=initIO unit='-' description='pne_brk_Axle2_torque_sns': IO_EBS_InputSignals.pne_brk_Axle2_torque_sns_0 [-]"; p187 "pne_brk_Axle3_BrakingForce_at8p5bar [N] (init) export=true name=pne_brk_Axle3_BrakingForce_at8p5bar prio=1 dataSetName=std dataClassType=initIO dataClassName=initIO unit=N description='pne_brk_Axle3_BrakingForce_at8p5bar [N] (init)': IO_EBS_InputSignals.pne_brk_Axle3_BrakingForce_at8p5bar_0 [-]"; p188 "axle 3 left temperature of the friction area [degC] (init) export=true name=pne_brk_Axle3_left_Tinterior prio=1 dataSetName=std dataClassType=initIO dataClassName=initIO unit=degC description='axle 1 left inner temperature [degC] (init)': IO_EBS_InputSignals.pne_brk_Axle3_left_Tinterior_0 [-]"; p189 "axle 3 right temperature of the friction area [degC] (init) export=true name=pne_brk_Axle3_right_Tinterior prio=1 dataSetName=std dataClassType=initIO dataClassName=initIO unit=degC description='axle 1 right inner temperature [degC] (init)': IO_EBS_InputSignals.pne_brk_Axle3_right_Tinterior_0 [-]"; p190 "pne_brk_Axle3_torque_sns export=true name=pne_brk_Axle3_torque_sns prio=1 dataSetName=std dataClassType=initIO dataClassName=initIO unit='-' description='pne_brk_Axle3_torque_sns': IO_EBS_InputSignals.pne_brk_Axle3_torque_sns_0 [-]"; p191 "pne_brk_Axle4_BrakingForce_at8p5bar [N] (init) export=true name=pne_brk_Axle4_BrakingForce_at8p5bar prio=1 dataSetName=std dataClassType=initIO dataClassName=initIO unit=N description='pne_brk_Axle4_BrakingForce_at8p5bar [N] (init)': IO_EBS_InputSignals.pne_brk_Axle4_BrakingForce_at8p5bar_0 [-]"; p192 "axle 4 left temperature of the friction area [degC] (init) export=true name=pne_brk_Axle4_left_Tinterior prio=1 dataSetName=std dataClassType=initIO dataClassName=initIO unit=degC description='axle 1 left inner temperature [degC] (init)': IO_EBS_InputSignals.pne_brk_Axle4_left_Tinterior_0 [-]"; p193 "axle 4 right temperature of the friction area [degC] (init) export=true name=pne_brk_Axle4_right_Tinterior prio=1 dataSetName=std dataClassType=initIO dataClassName=initIO unit=degC description='axle 1 right inner temperature [degC] (init)': IO_EBS_InputSignals.pne_brk_Axle4_right_Tinterior_0 [-]"; p194 "pne_brk_Axle4_torque_sns export=true name=pne_brk_Axle4_torque_sns prio=1 dataSetName=std dataClassType=initIO dataClassName=initIO unit='-' description='pne_brk_Axle4_torque_sns': IO_EBS_InputSignals.pne_brk_Axle4_torque_sns_0 [-]"; p195 "Front axle: acting pressure export=true name=pne_brk_FrontAxle_pAct prio=1 dataSetName=std dataClassType=initIO dataClassName=initIO unit='bar' description='Front axle: acting pressure': IO_EBS_InputSignals.pne_brk_FrontAxle_pAct_0 [-]"; p196 "Rear axle left: acting pressure export=true name=pne_brk_RearAxle_left_pAct prio=1 dataSetName=std dataClassType=initIO dataClassName=initIO unit='bar' description='Rear axle left: acting pressure': IO_EBS_InputSignals.pne_brk_RearAxle_left_pAct_0 [-]"; p197 "Rear axle right: acting pressure export=true name=pne_brk_RearAxle_right_pAct prio=1 dataSetName=std dataClassType=initIO dataClassName=initIO unit='bar' description='Rear axle right: acting pressure': IO_EBS_InputSignals.pne_brk_RearAxle_right_pAct_0 [-]"; p198 "wheel speed additional left wheel export=true name=pne_brk_rotVel_al prio=1 dataSetName=std dataClassType=initIO dataClassName=initIO unit='-' description='wheel speed additional left wheel': IO_EBS_InputSignals.pne_brk_rotVel_al_0 [-]"; p199 "wheel speed additional right wheel export=true name=pne_brk_rotVel_ar prio=1 dataSetName=std dataClassType=initIO dataClassName=initIO unit='-' description='wheel speed additional right wheel': IO_EBS_InputSignals.pne_brk_rotVel_ar_0 [-]"; p200 "wheel speed front left wheel export=true name=pne_brk_rotVel_fl prio=1 dataSetName=std dataClassType=initIO dataClassName=initIO unit='-' description='wheel speed front left wheel': IO_EBS_InputSignals.pne_brk_rotVel_fl_0 [-]"; p201 "wheel speed front right wheel export=true name=pne_brk_rotVel_fr prio=1 dataSetName=std dataClassType=initIO dataClassName=initIO unit='-' description='wheel speed front right wheel': IO_EBS_InputSignals.pne_brk_rotVel_fr_0 [-]"; p202 "wheel speed rear left wheel export=true name=pne_brk_rotVel_rl prio=1 dataSetName=std dataClassType=initIO dataClassName=initIO unit='-' description='wheel speed rear left wheel': IO_EBS_InputSignals.pne_brk_rotVel_rl_0 [-]"; p203 "wheel speed rear right wheel export=true name=pne_brk_rotVel_rr prio=1 dataSetName=std dataClassType=initIO dataClassName=initIO unit='-' description='wheel speed rear right wheel': IO_EBS_InputSignals.pne_brk_rotVel_rr_0 [-]"; p204 "Front axle: acting pressure export=true name=pne_brk_TCV_pAct prio=1 dataSetName=std dataClassType=initIO dataClassName=initIO unit='bar' description='actual pressure TCV': IO_EBS_InputSignals.pne_brk_TCV_pAct_0 [-]"; p205 "pne_brk_Trailer02Axle1_BrakingForce_at8p5bar [N] (init) export=true name=pne_brk_Trailer02Axle1_BrakingForce_at8p5bar prio=1 dataSetName=std dataClassType=initIO dataClassName=initIO unit=N description='pne_brk_Trailer02Axle1_BrakingForce_at8p5bar [N] (init)': IO_EBS_InputSignals.pne_brk_Trailer02Axle1_BrakingForce_at8p5bar_0 [-]"; p206 "pne_brk_Trailer02Axle1_torque_sns (init) export=true name=pne_brk_Trailer02Axle1_torque_sns prio=1 dataSetName=std dataClassType=initIO dataClassName=initIO unit=kg description='pne_brk_Trailer02Axle1_torque_sns': IO_EBS_InputSignals.pne_brk_Trailer02Axle1_torque_sns_0 [-]"; p207 "pne_brk_Trailer02Axle2_BrakingForce_at8p5bar [N] (init) export=true name=pne_brk_Trailer02Axle2_BrakingForce_at8p5bar prio=1 dataSetName=std dataClassType=initIO dataClassName=initIO unit=N description='pne_brk_Trailer02Axle2_BrakingForce_at8p5bar [N] (init)': IO_EBS_InputSignals.pne_brk_Trailer02Axle2_BrakingForce_at8p5bar_0 [-]"; p208 "pne_brk_Trailer02Axle2_torque_sns (init) export=true name=pne_brk_Trailer02Axle2_torque_sns prio=1 dataSetName=std dataClassType=initIO dataClassName=initIO unit=kg description='pne_brk_Trailer02Axle2_torque_sns': IO_EBS_InputSignals.pne_brk_Trailer02Axle2_torque_sns_0 [-]"; p209 "pne_brk_Trailer02Axle3_BrakingForce_at8p5bar [N] (init) export=true name=pne_brk_Trailer02Axle3_BrakingForce_at8p5bar prio=1 dataSetName=std dataClassType=initIO dataClassName=initIO unit=N description='pne_brk_Trailer02Axle3_BrakingForce_at8p5bar [N] (init)': IO_EBS_InputSignals.pne_brk_Trailer02Axle3_BrakingForce_at8p5bar_0 [-]"; p210 "pne_brk_Trailer02Axle3_torque_sns (init) export=true name=pne_brk_Trailer02Axle3_torque_sns prio=1 dataSetName=std dataClassType=initIO dataClassName=initIO unit=kg description='pne_brk_Trailer02Axle3_torque_sns': IO_EBS_InputSignals.pne_brk_Trailer02Axle3_torque_sns_0 [-]"; p211 "pne_brk_Trailer02Axle4_BrakingForce_at8p5bar [N] (init) export=true name=pne_brk_Trailer02Axle4_BrakingForce_at8p5bar prio=1 dataSetName=std dataClassType=initIO dataClassName=initIO unit=N description='pne_brk_Trailer02Axle4_BrakingForce_at8p5bar [N] (init)': IO_EBS_InputSignals.pne_brk_Trailer02Axle4_BrakingForce_at8p5bar_0 [-]"; p212 "pne_brk_Trailer02Axle4_torque_sns (init) export=true name=pne_brk_Trailer02Axle4_torque_sns prio=1 dataSetName=std dataClassType=initIO dataClassName=initIO unit=kg description='pne_brk_Trailer02Axle4_torque_sns': IO_EBS_InputSignals.pne_brk_Trailer02Axle4_torque_sns_0 [-]"; p213 "pne_brk_Trailer02Axle5_BrakingForce_at8p5bar [N] (init) export=true name=pne_brk_Trailer02Axle5_BrakingForce_at8p5bar prio=1 dataSetName=std dataClassType=initIO dataClassName=initIO unit=N description='pne_brk_Trailer02Axle5_BrakingForce_at8p5bar [N] (init)': IO_EBS_InputSignals.pne_brk_Trailer02Axle5_BrakingForce_at8p5bar_0 [-]"; p214 "pne_brk_Trailer02Axle5_torque_sns (init) export=true name=pne_brk_Trailer02Axle5_torque_sns prio=1 dataSetName=std dataClassType=initIO dataClassName=initIO unit=kg description='pne_brk_Trailer02Axle5_torque_sns': IO_EBS_InputSignals.pne_brk_Trailer02Axle5_torque_sns_0 [-]"; p215 "pne_brk_Trailer02Axle6_BrakingForce_at8p5bar [N] (init) export=true name=pne_brk_Trailer02Axle6_BrakingForce_at8p5bar prio=1 dataSetName=std dataClassType=initIO dataClassName=initIO unit=N description='pne_brk_Trailer02Axle6_BrakingForce_at8p5bar [N] (init)': IO_EBS_InputSignals.pne_brk_Trailer02Axle6_BrakingForce_at8p5bar_0 [-]"; p216 "pne_brk_Trailer02Axle6_torque_sns (init) export=true name=pne_brk_Trailer02Axle6_torque_sns prio=1 dataSetName=std dataClassType=initIO dataClassName=initIO unit=kg description='pne_brk_Trailer02Axle6_torque_sns': IO_EBS_InputSignals.pne_brk_Trailer02Axle6_torque_sns_0 [-]"; p217 "pne_brk_TrailerAxle1_BrakingForce_at8p5bar [N] (init) export=true name=pne_brk_TrailerAxle1_BrakingForce_at8p5bar prio=1 dataSetName=std dataClassType=initIO dataClassName=initIO unit=N description='pne_brk_TrailerAxle1_BrakingForce_at8p5bar [N] (init)': IO_EBS_InputSignals.pne_brk_TrailerAxle1_BrakingForce_at8p5bar_0 [-]"; p218 "pne_brk_TrailerAxle1_torque_sns export=true name=pne_brk_TrailerAxle1_torque_sns prio=1 dataSetName=std dataClassType=initIO dataClassName=initIO unit='-' description='pne_brk_TrailerAxle1_torque_sns': IO_EBS_InputSignals.pne_brk_TrailerAxle1_torque_sns_0 [-]"; p219 "pne_brk_TrailerAxle2_BrakingForce_at8p5bar [N] (init) export=true name=pne_brk_TrailerAxle2_BrakingForce_at8p5bar prio=1 dataSetName=std dataClassType=initIO dataClassName=initIO unit=N description='pne_brk_TrailerAxle2_BrakingForce_at8p5bar [N] (init)': IO_EBS_InputSignals.pne_brk_TrailerAxle2_BrakingForce_at8p5bar_0 [-]"; p220 "pne_brk_TrailerAxle2_torque_sns export=true name=pne_brk_TrailerAxle2_torque_sns prio=1 dataSetName=std dataClassType=initIO dataClassName=initIO unit='-' description='pne_brk_TrailerAxle2_torque_sns': IO_EBS_InputSignals.pne_brk_TrailerAxle2_torque_sns_0 [-]"; p221 "pne_brk_TrailerAxle3_BrakingForce_at8p5bar [N] (init) export=true name=pne_brk_TrailerAxle3_BrakingForce_at8p5bar prio=1 dataSetName=std dataClassType=initIO dataClassName=initIO unit=N description='pne_brk_TrailerAxle3_BrakingForce_at8p5bar [N] (init)': IO_EBS_InputSignals.pne_brk_TrailerAxle3_BrakingForce_at8p5bar_0 [-]"; p222 "pne_brk_TrailerAxle3_torque_sns export=true name=pne_brk_TrailerAxle3_torque_sns prio=1 dataSetName=std dataClassType=initIO dataClassName=initIO unit='-' description='pne_brk_TrailerAxle3_torque_sns': IO_EBS_InputSignals.pne_brk_TrailerAxle3_torque_sns_0 [-]"; p223 "PwrVehWeight_Cval (init) export=true name=PwrVehWeight_Cval prio=1 dataSetName=std dataClassType=initIO dataClassName=initIO unit=kg description='PwrVehWeight_Cval': IO_EBS_InputSignals.PwrVehWeight_Cval_0 [-]"; p224 "Retarder Percent Torque Actual 2 Current value from CPC3 export=true name=RetPctTrqActl2_Cval_CPC3 prio=1 dataSetName=std dataClassType=initIO dataClassName=initIO unit='-' description='Retarder Percent Torque Actual 2 Current value from CPC3': IO_EBS_InputSignals.RetPctTrqActl2_Cval_CPC3_0 [-]"; p225 "Retarder Reference Torque Value export=true name=RetRefTrq_Cval prio=1 dataSetName=std dataClassType=initIO dataClassName=initIO unit='-' description='Retarder Reference Torque Value': IO_EBS_InputSignals.RetRefTrq_Cval_0 [-]"; p226 "Road Curvature Current value, 65535 SNA; export=true name=RoadCurv_Cval prio=1 dataSetName=std dataClassType=initIO dataClassName=initIO unit='1/km' description='Road Curvature Current value, 65535 SNA;': IO_EBS_InputSignals.RoadCurv_Cval_0 [-]"; p227 "ROP_BrkCtrlActv2_Stat export=true name=ROP_BrkCtrlActv2_Stat prio=1 dataSetName=std dataClassType=initIO dataClassName=initIO unit='-' description='ROP_BrkCtrlActv2_Stat': IO_EBS_InputSignals.ROP_BrkCtrlActv2_Stat_0 [-]"; p228 "ROP_EngCtrlActv2_Stat export=true name=ROP_EngCtrlActv2_Stat prio=1 dataSetName=std dataClassType=initIO dataClassName=initIO unit='-' description='ROP_EngCtrlActv2_Stat': IO_EBS_InputSignals.ROP_EngCtrlActv2_Stat_0 [-]"; p229 "sAccel_X_Cval_SBSP export=true name=sAccel_X_Cval_SBSP prio=1 dataSetName=std dataClassType=initIO dataClassName=initIO unit='m/s^2' description='sAccel_X_Cval_SBSP': IO_EBS_InputSignals.sAccel_X_Cval_SBSP_0 [-]"; p230 "sAccel_Y_Cval_SBSP export=true name=sAccel_Y_Cval_SBSP prio=1 dataSetName=std dataClassType=initIO dataClassName=initIO unit='m/s^2' description='sAccel_Y_Cval_SBSP': IO_EBS_InputSignals.sAccel_Y_Cval_SBSP_0 [-]"; p231 "sAddInfoVehSped_Cval_SBSP export=true name=sAddInfoVehSped_Cval_SBSP prio=1 dataSetName=std dataClassType=initIO dataClassName=initIO unit='-' description='sAddInfoVehSped_Cval_SBSP': IO_EBS_InputSignals.sAddInfoVehSped_Cval_SBSP_0 [-]"; p232 "sBrkPdlPosn3_Cval_SBSP export=true name=sBrkPdlPosn3_Cval_SBSP prio=1 dataSetName=std dataClassType=initIO dataClassName=initIO unit='%' description='sBrkPdlPosn3_Cval_SBSP': IO_EBS_InputSignals.sBrkPdlPosn3_Cval_SBSP_0 [-]"; p233 "sBS_Brk_Cval_SBSP export=true name=sBS_Brk_Cval_SBSP prio=1 dataSetName=std dataClassType=initIO dataClassName=initIO unit='%' description='sBS_Brk_Cval_SBSP': IO_EBS_InputSignals.sBS_Brk_Cval_SBSP_0 [-]"; p234 "sBS_CS_Acc_Stat_SBSP export=true name=sBS_CS_Acc_Stat_SBSP prio=1 dataSetName=std dataClassType=initIO dataClassName=initIO unit='-' description='sBS_CS_Acc_Stat_SBSP': IO_EBS_InputSignals.sBS_CS_Acc_Stat_SBSP_0 [-]"; p235 "sBS_CS_RqPerf2_Stat_SBSP export=true name=sBS_CS_RqPerf2_Stat_SBSP prio=1 dataSetName=std dataClassType=initIO dataClassName=initIO unit='-' description='sBS_CS_RqPerf2_Stat_SBSP': IO_EBS_InputSignals.sBS_CS_RqPerf2_Stat_SBSP_0 [-]"; p236 "sBS_CS_RqPerf_Stat_SBSP export=true name=sBS_CS_RqPerf_Stat_SBSP prio=1 dataSetName=std dataClassType=initIO dataClassName=initIO unit='-' description='sBS_CS_RqPerf_Stat_SBSP': IO_EBS_InputSignals.sBS_CS_RqPerf_Stat_SBSP_0 [-]"; p237 "sBS_CSCPC_Acc_Stat_SBSP export=true name=sBS_CSCPC_Acc_Stat_SBSP prio=1 dataSetName=std dataClassType=initIO dataClassName=initIO unit='-' description='sBS_CSCPC_Acc_Stat_SBSP': IO_EBS_InputSignals.sBS_CSCPC_Acc_Stat_SBSP_0 [-]"; p238 "sBS_HB_Acc_Stat_SBSP export=true name=sBS_HB_Acc_Stat_SBSP prio=1 dataSetName=std dataClassType=initIO dataClassName=initIO unit='-' description='sBS_HB_Acc_Stat_SBSP': IO_EBS_InputSignals.sBS_HB_Acc_Stat_SBSP_0 [-]"; p239 "sBS_HB_RqPerf_Stat_SBSP export=true name=sBS_HB_RqPerf_Stat_SBSP prio=1 dataSetName=std dataClassType=initIO dataClassName=initIO unit='-' description='sBS_HB_RqPerf_Stat_SBSP': IO_EBS_InputSignals.sBS_HB_RqPerf_Stat_SBSP_0 [-]"; p240 "sBS_HBCPC_Acc_Stat_SBSP export=true name=sBS_HBCPC_Acc_Stat_SBSP prio=1 dataSetName=std dataClassType=initIO dataClassName=initIO unit='-' description='sBS_HBCPC_Acc_Stat_SBSP': IO_EBS_InputSignals.sBS_HBCPC_Acc_Stat_SBSP_0 [-]"; p241 "sBS_HBCPC_RqPerf_Stat_SBSP export=true name=sBS_HBCPC_RqPerf_Stat_SBSP prio=1 dataSetName=std dataClassType=initIO dataClassName=initIO unit='-' description='sBS_HBCPC_RqPerf_Stat_SBSP': IO_EBS_InputSignals.sBS_HBCPC_RqPerf_Stat_SBSP_0 [-]"; p242 "sBS_SS_Acc_Stat_SBSP export=true name=sBS_SS_Acc_Stat_SBSP prio=1 dataSetName=std dataClassType=initIO dataClassName=initIO unit='-' description='sBS_SS_Acc_Stat_SBSP': IO_EBS_InputSignals.sBS_SS_Acc_Stat_SBSP_0 [-]"; p243 "sBS_SS_RqPerf_Stat_SBSP export=true name=sBS_SS_RqPerf_Stat_SBSP prio=1 dataSetName=std dataClassType=initIO dataClassName=initIO unit='-' description='sBS_SS_RqPerf_Stat_SBSP': IO_EBS_InputSignals.sBS_SS_RqPerf_Stat_SBSP_0 [-]"; p244 "sConfLatAccel_SBSP export=true name=sConfLatAccel_SBSP prio=1 dataSetName=std dataClassType=initIO dataClassName=initIO unit='%' description='sConfLatAccel_SBSP': IO_EBS_InputSignals.sConfLatAccel_SBSP_0 [-]"; p245 "sConfLgtAccel_SBSP export=true name=sConfLgtAccel_SBSP prio=1 dataSetName=std dataClassType=initIO dataClassName=initIO unit='%' description='sConfLgtAccel_SBSP': IO_EBS_InputSignals.sConfLgtAccel_SBSP_0 [-]"; p246 "sConfYawRate_SBSP export=true name=sConfYawRate_SBSP prio=1 dataSetName=std dataClassType=initIO dataClassName=initIO unit='%' description='sConfYawRate_SBSP': IO_EBS_InputSignals.sConfYawRate_SBSP_0 [-]"; p247 "sEBS_BrkSw2_Rq_SBSP export=true name=sEBS_BrkSw2_Rq_SBSP prio=1 dataSetName=std dataClassType=initIO dataClassName=initIO unit='-' description='sEBS_BrkSw2_Rq_SBSP': IO_EBS_InputSignals.sEBS_BrkSw2_Rq_SBSP_0 [-]"; p248 "Full Braking Allowed state export=true name=sFullBrkAllow_Stat_SBSP prio=1 dataSetName=std dataClassType=initIO dataClassName=initIO unit='-' description='Full Braking Allowed state': IO_EBS_InputSignals.sFullBrkAllow_Stat_SBSP_0 [-]"; p249 "wheel speed of the truck front left wheel [km/h] export=true name=SpdFtAxleLtWhl_Cval prio=1 dataSetName=std dataClassType=initIO dataClassName=initIO unit='km/h' description='wheel speed of the truck front left wheel [km/h]': IO_EBS_InputSignals.SpdFtAxleLtWhl_Cval_0 [-]"; p250 "wheel speed of the truck front left wheel [km/h] export=true name=SpdFtAxleLtWhl_Cval_SBSP prio=1 dataSetName=std dataClassType=initIO dataClassName=initIO unit='km/h' description='wheel speed of the truck front left wheel [km/h]': IO_EBS_InputSignals.SpdFtAxleLtWhl_Cval_SBSP_0 [-]"; p251 "wheel speed of the truck front right wheel [km/h] export=true name=SpdFtAxleRtWhl_Cval prio=1 dataSetName=std dataClassType=initIO dataClassName=initIO unit='km/h' description='wheel speed of the truck front right wheel [km/h]': IO_EBS_InputSignals.SpdFtAxleRtWhl_Cval_0 [-]"; p252 "wheel speed of the truck front right wheel [km/h] export=true name=SpdFtAxleRtWhl_Cval_SBSP prio=1 dataSetName=std dataClassType=initIO dataClassName=initIO unit='km/h' description='wheel speed of the truck front right wheel [km/h]': IO_EBS_InputSignals.SpdFtAxleRtWhl_Cval_SBSP_0 [-]"; p253 "wheel speed of the truck rear left wheel [km/h] export=true name=SpdR_AxleLtWhl_Cval prio=1 dataSetName=std dataClassType=initIO dataClassName=initIO unit='km/h' description='wheel speed of the truck rear left wheel [km/h]': IO_EBS_InputSignals.SpdR_AxleLtWhl_Cval_0 [-]"; p254 "wheel speed of the truck rear left wheel [km/h] export=true name=SpdR_AxleLtWhl_Cval_SBSP prio=1 dataSetName=std dataClassType=initIO dataClassName=initIO unit='km/h' description='wheel speed of the truck rear left wheel [km/h]': IO_EBS_InputSignals.SpdR_AxleLtWhl_Cval_SBSP_0 [-]"; p255 "wheel speed of the truck rear right wheel [km/h] export=true name=SpdR_AxleRtWhl_Cval prio=1 dataSetName=std dataClassType=initIO dataClassName=initIO unit='km/h' description='wheel speed of the truck rear right wheel [km/h]': IO_EBS_InputSignals.SpdR_AxleRtWhl_Cval_0 [-]"; p256 "wheel speed of the truck rear right wheel [km/h] export=true name=SpdR_AxleRtWhl_Cval_SBSP prio=1 dataSetName=std dataClassType=initIO dataClassName=initIO unit='km/h' description='wheel speed of the truck rear right wheel [km/h]': IO_EBS_InputSignals.SpdR_AxleRtWhl_Cval_SBSP_0 [-]"; p257 "SrcAdrBrkCtrlDev_Cval export=true name=SrcAdrBrkCtrlDev_Cval prio=1 dataSetName=std dataClassType=initIO dataClassName=initIO unit='-' description='SrcAdrBrkCtrlDev_Cval': IO_EBS_InputSignals.SrcAdrBrkCtrlDev_Cval_0 [-]"; p258 "SrcAdrBrkCtrlDev_Cval_SBSP export=true name=SrcAdrBrkCtrlDev_Cval_SBSP prio=1 dataSetName=std dataClassType=initIO dataClassName=initIO unit='-' description='SrcAdrBrkCtrlDev_Cval_SBSP': IO_EBS_InputSignals.SrcAdrBrkCtrlDev_Cval_SBSP_0 [-]"; p259 "sSpdFtAxleLtWhl_Cval_SBSP export=true name=sSpdFtAxleLtWhl_Cval_SBSP prio=1 dataSetName=std dataClassType=initIO dataClassName=initIO unit='km/h' description='sSpdFtAxleLtWhl_Cval_SBSP': IO_EBS_InputSignals.sSpdFtAxleLtWhl_Cval_SBSP_0 [-]"; p260 "sSpdFtAxleRtWhl_Cval_SBSP export=true name=sSpdFtAxleRtWhl_Cval_SBSP prio=1 dataSetName=std dataClassType=initIO dataClassName=initIO unit='km/h' description='sSpdFtAxleRtWhl_Cval_SBSP': IO_EBS_InputSignals.sSpdFtAxleRtWhl_Cval_SBSP_0 [-]"; p261 "sSpdR_AxleLtWhl_Cval_SBSP export=true name=sSpdR_AxleLtWhl_Cval_SBSP prio=1 dataSetName=std dataClassType=initIO dataClassName=initIO unit='km/h' description='sSpdR_AxleLtWhl_Cval_SBSP': IO_EBS_InputSignals.sSpdR_AxleLtWhl_Cval_SBSP_0 [-]"; p262 "sSpdR_AxleRtWhl_Cval_SBSP export=true name=sSpdR_AxleRtWhl_Cval_SBSP prio=1 dataSetName=std dataClassType=initIO dataClassName=initIO unit='km/h' description='sSpdR_AxleRtWhl_Cval_SBSP': IO_EBS_InputSignals.sSpdR_AxleRtWhl_Cval_SBSP_0 [-]"; p263 "sSrcAdrBrkCtrlDev_Cval_SBSP export=true name=sSrcAdrBrkCtrlDev_Cval_SBSP prio=1 dataSetName=std dataClassType=initIO dataClassName=initIO unit='-' description='sSrcAdrBrkCtrlDev_Cval_SBSP': IO_EBS_InputSignals.sSrcAdrBrkCtrlDev_Cval_SBSP_0 [-]"; p264 "sStandstill_Dtct_Stat_SBSP export=true name=sStandstill_Dtct_Stat_SBSP prio=1 dataSetName=std dataClassType=initIO dataClassName=initIO unit='-' description='sStandstill_Dtct_Stat_SBSP': IO_EBS_InputSignals.sStandstill_Dtct_Stat_SBSP_0 [-]"; p265 "Standstill_Dtct_Stat_SBSP (init) export=true name=Standstill_Dtct_Stat_SBSP prio=1 dataSetName=std dataClassType=initIO dataClassName=initIO unit='-' description='Standstill_Dtct_Stat_SBSP': IO_EBS_InputSignals.Standstill_Dtct_Stat_SBSP_0 [-]"; p266 "sTrlrAbsOper_Stat export=true name=sTrlrAbsOper_Stat prio=1 dataSetName=std dataClassType=initIO dataClassName=initIO unit='-' description='sTrlrAbsOper_Stat': IO_EBS_InputSignals.sTrlrAbsOper_Stat_0 [-]"; p267 "sTrlrEstm_Stat_SBSP export=true name=sTrlrEstm_Stat_SBSP prio=1 dataSetName=std dataClassType=initIO dataClassName=initIO unit='-' description='sTrlrEstm_Stat_SBSP': IO_EBS_InputSignals.sTrlrEstm_Stat_SBSP_0 [-]"; p268 "sVehSpd_Cval_SBSP export=true name=sVehSpd_Cval_SBSP prio=1 dataSetName=std dataClassType=initIO dataClassName=initIO unit='km/h' description='sVehSpd_Cval_SBSP': IO_EBS_InputSignals.sVehSpd_Cval_SBSP_0 [-]"; p269 "sXBR_AccelLim_Stat_SBSP export=true name=sXBR_AccelLim_Stat_SBSP prio=1 dataSetName=std dataClassType=initIO dataClassName=initIO unit='m/s^2' description='sXBR_AccelLim_Stat_SBSP': IO_EBS_InputSignals.sXBR_AccelLim_Stat_SBSP_0 [-]"; p270 "sXBR_ActCtrl_Stat_SBSP export=true name=sXBR_ActCtrl_Stat_SBSP prio=1 dataSetName=std dataClassType=initIO dataClassName=initIO unit='-' description='sXBR_ActCtrl_Stat_SBSP': IO_EBS_InputSignals.sXBR_ActCtrl_Stat_SBSP_0 [-]"; p271 "sXBR_Sys_Stat_SBSP export=true name=sXBR_Sys_Stat_SBSP prio=1 dataSetName=std dataClassType=initIO dataClassName=initIO unit='-' description='sXBR_Sys_Stat_SBSP': IO_EBS_InputSignals.sXBR_Sys_Stat_SBSP_0 [-]"; p272 "sYawRateCorr_Cval_SBSP export=true name=sYawRateCorr_Cval_SBSP prio=1 dataSetName=std dataClassType=initIO dataClassName=initIO unit='rad/s' description='sYawRateCorr_Cval_SBSP': IO_EBS_InputSignals.sYawRateCorr_Cval_SBSP_0 [-]"; p273 "TrctrAbsOper_Stat export=true name=TrctrAbsOper_Stat prio=1 dataSetName=std dataClassType=initIO dataClassName=initIO unit='-' description='TrctrAbsOper_Stat': IO_EBS_InputSignals.TrctrAbsOper_Stat_0 [-]"; p274 "TrlrAbsOper_Stat (init) Trailer Estimation Current state BS 0-OFF, 1-ABS_SIMUL, 2-FULL, 3-SNA export=true name=TrlrAbsOper_Stat prio=1 dataSetName=std dataClassType=initIO dataClassName=initIO unit='-' description='Trailer Estimation Current state BS 0-OFF, 1-ABS_SIMUL, 2-FULL, 3-SNA': IO_EBS_InputSignals.TrlrAbsOper_Stat_0 [-]"; p275 "TrlrEstm_Stat_SBSP (init) export=true name=TrlrEstm_Stat_SBSP prio=1 dataSetName=std dataClassType=initIO dataClassName=initIO unit='-' description='TrlrEstm_Stat_SBSP': IO_EBS_InputSignals.TrlrEstm_Stat_SBSP_0 [-]"; p276 "TrqConv_Cval_PT export=true name=TrqConv_Cval_PT prio=1 dataSetName=std dataClassType=initIO dataClassName=initIO unit='-' description='TrqConv_Cval_PT': IO_EBS_InputSignals.TrqConv_Cval_PT_0 [-]"; p277 "Gearbox InputShaft Speed RPM Current value from CPC export=true name=TxInShaftSpd_Cval_CPC prio=1 dataSetName=std dataClassType=initIO dataClassName=initIO unit='-' description='Gearbox InputShaft Speed RPM Current value from CPC': IO_EBS_InputSignals.TxInShaftSpd_Cval_CPC_0 [-]"; p278 "Tyre Correction Value Front Axel left, 255 SNA; export=true name=TyreCorrLtFA_Cval prio=1 dataSetName=std dataClassType=initIO dataClassName=initIO unit='%' description='Tyre Correction Value Front Axel left, 255 SNA;': IO_EBS_InputSignals.TyreCorrLtFA_Cval_0 [-]"; p279 "Tyre Correction Value Rear Axel left, 255 SNA; export=true name=TyreCorrLtRA_Cval prio=1 dataSetName=std dataClassType=initIO dataClassName=initIO unit='%' description='Tyre Correction Value Rear Axel left, 255 SNA;': IO_EBS_InputSignals.TyreCorrLtRA_Cval_0 [-]"; p280 "Tyre Correction Value Front Axel Right, 255 SNA; export=true name=TyreCorrRtFA_Cval prio=1 dataSetName=std dataClassType=initIO dataClassName=initIO unit='%' description='Tyre Correction Value Front Axel Right, 255 SNA;': IO_EBS_InputSignals.TyreCorrRtFA_Cval_0 [-]"; p281 "Tyre Correction Value Rear Axel right, 255 SNA; export=true name=TyreCorrRtRA_Cval prio=1 dataSetName=std dataClassType=initIO dataClassName=initIO unit='%' description='Tyre Correction Value Rear Axel right, 255 SNA;': IO_EBS_InputSignals.TyreCorrRtRA_Cval_0 [-]"; p282 "Tyre Rolling Circumference Front Axel, 255 SNA; export=true name=TyreRollCircumFA_Cval prio=1 dataSetName=std dataClassType=initIO dataClassName=initIO unit='mm' description='Tyre Rolling Circumference Front Axel, 255 SNA;': IO_EBS_InputSignals.TyreRollCircumFA_Cval_0 [-]"; p283 "Tyre Rolling Circumference Rear Axel, 255 SNA; export=true name=TyreRollCircumRA_Cval prio=1 dataSetName=std dataClassType=initIO dataClassName=initIO unit='mm' description='Tyre Rolling Circumference Rear Axel, 255 SNA;': IO_EBS_InputSignals.TyreRollCircumRA_Cval_0 [-]"; p284 "Trailer Velocity export=true name=VehSpd1_Cval_Trlr prio=1 dataSetName=std dataClassType=initIO dataClassName=initIO unit='-' description='Trailer Velocity': IO_EBS_InputSignals.VehSpd1_Cval_Trlr_0 [-]"; p285 "speed of the truck [km/h] export=true name=VehSpd_Cval_BS prio=1 dataSetName=std dataClassType=initIO dataClassName=initIO unit='km/h' description='speed of the truck [km/h]': IO_EBS_InputSignals.VehSpd_Cval_BS_0 [-]"; p286 "VehSpd_Cval_SBSP (init) export=true name=VehSpd_Cval_SBSP prio=1 dataSetName=std dataClassType=initIO dataClassName=initIO unit='km/h' description='VehSpd_Cval_SBSP': IO_EBS_InputSignals.VehSpd_Cval_SBSP_0 [-]"; p287 "XBR_AccelLim_Stat_BS export=true name=XBR_AccelLim_Stat_BS prio=1 dataSetName=std dataClassType=initIO dataClassName=initIO unit=m/s^2 description='XBR_AccelLim_Stat_BS': IO_EBS_InputSignals.XBR_AccelLim_Stat_BS_0 [-]"; p288 "XBR_AccelLim_Stat_SBSP export=true name=XBR_AccelLim_Stat_SBSP prio=1 dataSetName=std dataClassType=initIO dataClassName=initIO unit=m/s^2 description='XBR_AccelLim_Stat_SBSP': IO_EBS_InputSignals.XBR_AccelLim_Stat_SBSP_0 [-]"; p289 "XBR_ActCtrl_Stat_SBSP export=true name=XBR_ActCtrl_Stat_SBSP prio=1 dataSetName=std dataClassType=initIO dataClassName=initIO unit='-' description='XBR_ActCtrl_Stat_SBSP': IO_EBS_InputSignals.XBR_ActCtrl_Stat_SBSP_0 [-]"; p290 "XBR_CtrlMode_Stat_CPC5ce export=true name=XBR_CtrlMode_Stat_CPC5ce prio=1 dataSetName=std dataClassType=initIO dataClassName=initIO unit='-' description='XBR_CtrlMode_Stat_CPC5ce': IO_EBS_InputSignals.XBR_CtrlMode_Stat_CPC5ce_0 [-]"; p291 "XBR_CtrlMode_Stat_VRDU export=true name=XBR_CtrlMode_Stat_VRDU prio=1 dataSetName=std dataClassType=initIO dataClassName=initIO unit='-' description='XBR_CtrlMode_Stat_VRDU': IO_EBS_InputSignals.XBR_CtrlMode_Stat_VRDU_0 [-]"; p292 "XBR_EBI_Stat_VRDU export=true name=XBR_EBI_Stat_VRDU prio=1 dataSetName=std dataClassType=initIO dataClassName=initIO unit='-' description='XBR_EBI_Stat_VRDU': IO_EBS_InputSignals.XBR_EBI_Stat_VRDU_0 [-]"; p293 "XBR_Prio_Stat_CPC5ce export=true name=XBR_Prio_Stat_CPC5ce prio=1 dataSetName=std dataClassType=initIO dataClassName=initIO unit='-' description='XBR_Prio_Stat_CPC5ce': IO_EBS_InputSignals.XBR_Prio_Stat_CPC5ce_0 [-]"; p294 "XBR_Prio_Stat_VRDU export=true name=XBR_Prio_Stat_VRDU prio=1 dataSetName=std dataClassType=initIO dataClassName=initIO unit='-' description='XBR_Prio_Stat_VRDU': IO_EBS_InputSignals.XBR_Prio_Stat_VRDU_0 [-]"; p295 "XBR_Sys_Stat_SBSP export=true name=XBR_Sys_Stat_SBSP prio=1 dataSetName=std dataClassType=initIO dataClassName=initIO unit='-' description='XBR_Sys_Stat_SBSP': IO_EBS_InputSignals.XBR_Sys_Stat_SBSP_0 [-]"; p296 "YawRateCorr_Cval_SBSP export=true name=YawRateCorr_Cval_SBSP prio=1 dataSetName=std dataClassType=initIO dataClassName=initIO unit='rad/s' description='YawRateCorr_Cval_SBSP': IO_EBS_InputSignals.YawRateCorr_Cval_SBSP_0 [-]"; p297 "YC_BrkCtrlActv2_Stat export=true name=YC_BrkCtrlActv2_Stat prio=1 dataSetName=std dataClassType=initIO dataClassName=initIO unit='-' description='YC_BrkCtrlActv2_Stat': IO_EBS_InputSignals.YC_BrkCtrlActv2_Stat_0 [-]"; p298 "YC_EngCtrlActv2_Stat export=true name=YC_EngCtrlActv2_Stat prio=1 dataSetName=std dataClassType=initIO dataClassName=initIO unit='-' description='YC_EngCtrlActv2_Stat': IO_EBS_InputSignals.YC_EngCtrlActv2_Stat_0 [-]"; p299 "Nominal InputShaft Displacement [-] export=true name=zSoll_dx_xAxis_nom prio=1 dataSetName=ebs_dummy dataClassType=main dataClassName=main  unit='-' description='Nominal InputShaft Displacement [-]': BWG.zSoll_dx_xAxis_nom [-]"; p300 "Nominal InputShaft Displacement [-] export=true name=zSoll_dx_yAxis_nom prio=1 dataSetName=ebs_dummy dataClassType=main dataClassName=main  unit='-' description='Nominal Deceleration Set Value [-]': BWG.zSoll_dx_yAxis_nom [-]"; p301 "Axle Loads Trailer export=true name=axleLoadTrailer02_kg prio=1 dataSetName=veh_dummy dataClassType=veh dataClassName=veh unit=kg description='Axle Loads Trailer02': eBS_veh_Param.axleLoadTrailer02_kg [-]"; p302 "Axle Loads Trailer export=true name=axleLoadTrailer_kg prio=1 dataSetName=veh_dummy dataClassType=veh dataClassName=veh unit=kg description='Axle Loads Trailer': eBS_veh_Param.axleLoadTrailer_kg [-]"; p303 "Axle Loads Vehicle export=true name=axleLoadVehicle_kg prio=1 dataSetName=veh_dummy dataClassType=veh dataClassName=veh unit=kg description='Axle Loads Vehicle': eBS_veh_Param.axleLoadVehicle_kg [-]"; p304 "Brake Circuit Configuration [A1, A2, A3, A4] (0-Dummy, 1-Front, 2-Rear, 3-Middle(Bus)) export=true name=brkCircuit prio=1 dataSetName=veh_dummy dataClassType=veh dataClassName=veh unit='-' description='Brake Circuit Configuration [A1, A2, A3, A4] (0-Dummy, 1-Front, 2-Rear, 3-Middle(Bus))': eBS_veh_Param.brkCircuit [-]"; p305 "Trailer Control Active / Trailer can brake {flag, x1, x2, x3, x4, x5, y1, y2, y3, y4, y5} (flag: 0 - no, 1- yes ALB lower limit, 2- yes ALB normal, 3- yes ALB upper limit , 4 - yes without ALB, 5 - with characteristics {{x1 ...x5},{y1...y5}) export=true name=flagTrailer02ControlActive prio=1 dataSetName=veh_dummy dataClassType=veh dataClassName=veh unit='-' description='Trailer Control Active / Trailer can brake {flag, x1, x2, x3, x4, x5, y1, y2, y3, y4, y5} (flag: 0 - no, 1- yes ALB lower limit, 2- yes ALB normal, 3- yes ALB upper limit , 4 - yes without ALB, 5 - with characteristics {{x1 ...x5},{y1...y5})': eBS_veh_Param.flagTrailer02ControlActive [-]"; p306 "Trailer Control Active / Trailer can brake {flag, x1, x2, x3, x4, x5, y1, y2, y3, y4, y5} (flag: 0 - no, 1- yes ALB lower limit, 2- yes ALB normal, 3- yes ALB upper limit , 4 - yes without ALB, 5 - with characteristics {{x1 ...x5},{y1...y5}) export=true name=flagTrailerControlActive prio=1 dataSetName=veh_dummy dataClassType=veh dataClassName=veh unit='-' description='Trailer Control Active / Trailer can brake {flag, x1, x2, x3, x4, x5, y1, y2, y3, y4, y5} (flag: 0 - no, 1- yes ALB lower limit, 2- yes ALB normal, 3- yes ALB upper limit , 4 - yes without ALB, 5 - with characteristics {{x1 ...x5},{y1...y5})': eBS_veh_Param.flagTrailerControlActive [-]"; p307 "pAppCyl Tractor Axles [A1, A2, A3, A4] [bar] export=true name=pAppCyl_Tractor prio=1 dataSetName=veh_dummy dataClassType=veh dataClassName=veh unit='bar' description='pAppCyl Tractor Axles [A1, A2, A3, A4] [bar]': eBS_veh_Param.pAppCyl_Tractor [-]"; p308 "pAppCyl Trailer Axles [TA1, TA2, TA3] [bar] export=true name=pAppCyl_Trailer prio=1 dataSetName=veh_dummy dataClassType=veh dataClassName=veh unit='bar' description='pAppCyl Trailer Axles [TA1, TA2, TA3] [bar]': eBS_veh_Param.pAppCyl_Trailer [-]"; p309 "application pressure of trailer axles [A1, A2, A3, A4, A5, A6] [bar] export=true name=pAppCyl_Trailer02 prio=1 dataSetName=veh_dummy dataClassType=veh dataClassName=veh unit='bar' description='application pressure of trailer axles [A1, A2, A3, A4, A5, A6]  [bar]': eBS_veh_Param.pAppCyl_Trailer02 [-]"; p310 "rdyn's of Trailer02 [A1,A2,A3, A4, A5, A6] export=true name=rdynTrailer02 prio=1 dataSetName=veh_dummy dataClassType=veh dataClassName=veh unit=mm description='Trailer02 rDyn': eBS_veh_Param.rdynTrailer02 [-]"; p311 "Vehicle Speed Sensor Axle Position {A1,A2,A3,A4} (0-false,1-true)  export=true name=speedSensorPosnVeh prio=1 dataSetName=veh_dummy dataClassType=veh dataClassName=veh unit='' description='Vehicle Speed Sensor Axle Position {A1,A2,A3,A4} (0-false,1-true)': eBS_veh_Param.speedSensorPosnVeh [-]"
      mask help: Generated by SimulationX 4.0.5.60286 x64
      mask init:
      | if ~isempty(initCmd), try, evalin('base', initCmd); end, end
      mask Display: disp('ebs_rebuild_generic_std_sf'); port_label('input', 1, 'env_curv_pm'); port_label('input', 2, 'env_road_slope_pct'); port_label('input', 3, 'ActlEmotTrq_Cval'); port_label('input', 4, 'ActlEngPctTrq_Cval'); port_label('input', 5, 'ActlMaxAvlRetPctTrq_Cval_CPC3'); port_label('input', 6, 'aSbspVehBrkForce_Cmd_SDS'); port_label('input', 7, 'BrkPress_Rq'); port_label('input', 8, 'Clutch_Stat_CPC'); port_label('input', 9, 'EdrvRefTrq_Cval'); port_label('input', 10, 'EngPctTrqActl_Cval'); port_label('input', 11, 'EngRefTrq_Cval'); port_label('input', 12, 'EngRPM_Cval_CPC3'); port_label('input', 13, 'ExtAccel_Rq_CPC'); port_label('input', 14, 'ExtAccel_Rq_CPC5ce'); port_label('input', 15, 'ExtAccel_Rq_VRDU'); port_label('input', 16, 'ExtAccel_Rq_VRDU3'); port_label('input', 17, 'ExtBrkStat_Rq_CPC'); port_label('input', 18, 'ExtBrkStat_Rq_VRDU'); port_label('input', 19, 'HB_Rq_Stat_CPC'); port_label('input', 20, 'HB_Rq_Stat_VRDU'); port_label('input', 21, 'MinAvlEmotTrq_Cval_CPC'); port_label('input', 22, 'NomFrictEngPctTrq_Cval'); port_label('input', 23, 'PkBrk_Rq_VRDU'); port_label('input', 24, 'RetPctTrqActl2_Cval_CPC3'); port_label('input', 25, 'RetRefTrq_Cval'); port_label('input', 26, 'TrqConv_Cval_PT'); port_label('input', 27, 'TxInShaftSpd_Cval_CPC'); port_label('input', 28, 'VehSpd1_Cval_Trlr'); port_label('input', 29, 'XBR_CtrlMode_Stat_CPC5ce'); port_label('input', 30, 'XBR_CtrlMode_Stat_VRDU'); port_label('input', 31, 'XBR_EBI_Stat_VRDU'); port_label('input', 32, 'XBR_Prio_Stat_CPC5ce'); port_label('input', 33, 'XBR_Prio_Stat_VRDU'); port_label('input', 34, 'drv_BrkPdl_pos'); port_label('input', 35, 'drv_PkBrk'); port_label('input', 36, 'mec3d_ESCsens_gamma_rate'); port_label('input', 37, 'mec3d_ESCsens_y_acceleration'); port_label('input', 38, 'mec_veh_AxleLoad1'); port_label('input', 39, 'mec_veh_AxleLoad2'); port_label('input', 40, 'mec_veh_AxleLoad3'); port_label('input', 41, 'mec_veh_AxleLoad4'); port_label('input', 42, 'mec_veh_Trailer02AxleLoad1'); port_label('input', 43, 'mec_veh_Trailer02AxleLoad2'); port_label('input', 44, 'mec_veh_Trailer02AxleLoad3'); port_label('input', 45, 'mec_veh_Trailer02AxleLoad4'); port_label('input', 46, 'mec_veh_Trailer02AxleLoad5'); port_label('input', 47, 'mec_veh_Trailer02AxleLoad6'); port_label('input', 48, 'mec_veh_TrailerAxleLoad1'); port_label('input', 49, 'mec_veh_TrailerAxleLoad2'); port_label('input', 50, 'mec_veh_TrailerAxleLoad3'); port_label('input', 51, 'mec_veh_transVel'); port_label('input', 52, 'pne_brk_AdditionalAxle_left_pAct'); port_label('input', 53, 'pne_brk_AdditionalAxle_right_pAct'); port_label('input', 54, 'pne_brk_Axle1_BrakingForce_at8p5bar'); port_label('input', 55, 'pne_brk_Axle1_left_Tinterior'); port_label('input', 56, 'pne_brk_Axle1_right_Tinterior'); port_label('input', 57, 'pne_brk_Axle1_torque_sns'); port_label('input', 58, 'pne_brk_Axle2_BrakingForce_at8p5bar'); port_label('input', 59, 'pne_brk_Axle2_left_Tinterior'); port_label('input', 60, 'pne_brk_Axle2_right_Tinterior'); port_label('input', 61, 'pne_brk_Axle2_torque_sns'); port_label('input', 62, 'pne_brk_Axle3_BrakingForce_at8p5bar'); port_label('input', 63, 'pne_brk_Axle3_left_Tinterior'); port_label('input', 64, 'pne_brk_Axle3_right_Tinterior'); port_label('input', 65, 'pne_brk_Axle3_torque_sns'); port_label('input', 66, 'pne_brk_Axle4_BrakingForce_at8p5bar'); port_label('input', 67, 'pne_brk_Axle4_left_Tinterior'); port_label('input', 68, 'pne_brk_Axle4_right_Tinterior'); port_label('input', 69, 'pne_brk_Axle4_torque_sns'); port_label('input', 70, 'pne_brk_FrontAxle_pAct'); port_label('input', 71, 'pne_brk_RearAxle_left_pAct'); port_label('input', 72, 'pne_brk_RearAxle_right_pAct'); port_label('input', 73, 'pne_brk_rotVel_al'); port_label('input', 74, 'pne_brk_rotVel_ar'); port_label('input', 75, 'pne_brk_rotVel_fl'); port_label('input', 76, 'pne_brk_rotVel_fr'); port_label('input', 77, 'pne_brk_rotVel_rl'); port_label('input', 78, 'pne_brk_rotVel_rr'); port_label('input', 79, 'pne_brk_TCV_pAct'); port_label('input', 80, 'pne_brk_Trailer02Axle1_BrakingForce_at8p5bar'); port_label('input', 81, 'pne_brk_Trailer02Axle1_torque_sns'); port_label('input', 82, 'pne_brk_Trailer02Axle2_BrakingForce_at8p5bar'); port_label('input', 83, 'pne_brk_Trailer02Axle2_torque_sns'); port_label('input', 84, 'pne_brk_Trailer02Axle3_BrakingForce_at8p5bar'); port_label('input', 85, 'pne_brk_Trailer02Axle3_torque_sns'); port_label('input', 86, 'pne_brk_Trailer02Axle4_BrakingForce_at8p5bar'); port_label('input', 87, 'pne_brk_Trailer02Axle4_torque_sns'); port_label('input', 88, 'pne_brk_Trailer02Axle5_BrakingForce_at8p5bar'); port_label('input', 89, 'pne_brk_Trailer02Axle5_torque_sns'); port_label('input', 90, 'pne_brk_Trailer02Axle6_BrakingForce_at8p5bar'); port_label('input', 91, 'pne_brk_Trailer02Axle6_torque_sns'); port_label('input', 92, 'pne_brk_TrailerAxle1_BrakingForce_at8p5bar'); port_label('input', 93, 'pne_brk_TrailerAxle1_torque_sns'); port_label('input', 94, 'pne_brk_TrailerAxle2_BrakingForce_at8p5bar'); port_label('input', 95, 'pne_brk_TrailerAxle2_torque_sns'); port_label('input', 96, 'pne_brk_TrailerAxle3_BrakingForce_at8p5bar'); port_label('input', 97, 'pne_brk_TrailerAxle3_torque_sns'); port_label('output', 1, 'ebs_AdditionalAxle_left_pDmd'); port_label('output', 2, 'ebs_AdditionalAxle_right_pDmd'); port_label('output', 3, 'ebs_ESCsens_y_acceleration'); port_label('output', 4, 'ebs_FrontAxle_left_pDmd'); port_label('output', 5, 'ebs_FrontAxle_right_pDmd'); port_label('output', 6, 'ebs_RearAxle_left_pDmd'); port_label('output', 7, 'ebs_RearAxle_right_pDmd'); port_label('output', 8, 'ebs_sBSP_stABSInValve_Addl_Left'); port_label('output', 9, 'ebs_sBSP_stABSInValve_Addl_Right'); port_label('output', 10, 'ebs_sBSP_stABSInValve_Front_Left'); port_label('output', 11, 'ebs_sBSP_stABSInValve_Front_Right'); port_label('output', 12, 'ebs_sBSP_stABSInValve_RCMax_Front'); port_label('output', 13, 'ebs_sBSP_stABSInValve_RCMax_Rear'); port_label('output', 14, 'ebs_sBSP_stABSInValve_Rear_Left'); port_label('output', 15, 'ebs_sBSP_stABSInValve_Rear_Right'); port_label('output', 16, 'ebs_sBSP_stABSOutValve_Addl_Left'); port_label('output', 17, 'ebs_sBSP_stABSOutValve_Addl_Right'); port_label('output', 18, 'ebs_sBSP_stABSOutValve_Front_Left'); port_label('output', 19, 'ebs_sBSP_stABSOutValve_Front_Right'); port_label('output', 20, 'ebs_sBSP_stABSOutValve_RCMax_Front'); port_label('output', 21, 'ebs_sBSP_stABSOutValve_RCMax_Rear'); port_label('output', 22, 'ebs_sBSP_stABSOutValve_Rear_Left'); port_label('output', 23, 'ebs_sBSP_stABSOutValve_Rear_Right'); port_label('output', 24, 'ebs_sBSP_stAPCVBuValve'); port_label('output', 25, 'ebs_sBSP_stAxmoBuValve'); port_label('output', 26, 'ebs_sBSP_stCMaxBuValve'); port_label('output', 27, 'ebs_TCV_pDmd'); port_label('output', 28, 'aAutoOpMd_Stat_SBSP'); port_label('output', 29, 'aBrkAirPressAA_Cval_SBSP'); port_label('output', 30, 'aBrkAirPressFA_Cval_SBSP'); port_label('output', 31, 'aBrkAirPressRA_Cval_SBSP'); port_label('output', 32, 'aBrkPdlPosn3_Cval_SBSP'); port_label('output', 33, 'aBrkTempFA_Cval_SBSP'); port_label('output', 34, 'aBrkTempIA_Cval_SBSP'); port_label('output', 35, 'aBrkTempRA_Cval_SBSP'); port_label('output', 36, 'ABS_Actv2_Stat'); port_label('output', 37, 'ABS_Actv_Stat'); port_label('output', 38, 'ABS_FullyOp_Stat'); port_label('output', 39, 'ABS_Trlr_Stat'); port_label('output', 40, 'Accel_X_Cval'); port_label('output', 41, 'Accel_X_Cval_SBSP'); port_label('output', 42, 'Accel_Y_Cval'); port_label('output', 43, 'Accel_Y_Cval_SBSP'); port_label('output', 44, 'AddInfoVehSped_Cval_SBSP'); port_label('output', 45, 'aGroCmbVehWeight_Cval_SBSP'); port_label('output', 46, 'aGroCmbVehWeightConf_SBSP'); port_label('output', 47, 'aStandstill_Dtct_Stat_SBSP'); port_label('output', 48, 'ATC_BrkCtrl_Stat'); port_label('output', 49, 'ATC_EngCtrl_Stat'); port_label('output', 50, 'ATC_InfoSgl_Stat'); port_label('output', 51, 'aTCV_Press_Cval_SBSP'); port_label('output', 52, 'aVehSpd_Cval_E2E_SBSP'); port_label('output', 53, 'aVehSpd_Cval_SBSP'); port_label('output', 54, 'BlockTend_Stat'); port_label('output', 55, 'BrkPdlPosn3_Cval'); port_label('output', 56, 'BrkPdlPosn3_Cval_SBSP'); port_label('output', 57, 'BrkPdlPosn_Cval'); port_label('output', 58, 'BS_Brk_Cval'); port_label('output', 59, 'BS_Brk_Cval_SBSP'); port_label('output', 60, 'BS_CS_Acc_Stat'); port_label('output', 61, 'BS_CS_Acc_Stat_SBSP'); port_label('output', 62, 'BS_CS_RqPerf2_Stat'); port_label('output', 63, 'BS_CS_RqPerf2_Stat_SBSP'); port_label('output', 64, 'BS_CS_RqPerf_Stat_SBSP'); port_label('output', 65, 'BS_CSCPC_Acc_Stat'); port_label('output', 66, 'BS_CSCPC_Acc_Stat_SBSP'); port_label('output', 67, 'BS_CSCPC_Intf_Stat'); port_label('output', 68, 'BS_CSCPC_RqPerf_Stat'); port_label('output', 69, 'BS_HB_Acc_Stat_SBSP'); port_label('output', 70, 'BS_HB_RqPerf_Stat'); port_label('output', 71, 'BS_HB_RqPerf_Stat_SBSP'); port_label('output', 72, 'BS_HBCPC_Acc_Stat_SBSP'); port_label('output', 73, 'BS_HBCPC_RqPerf_Stat_SBSP'); port_label('output', 74, 'BS_RoadIncln_Cval'); port_label('output', 75, 'BS_SS_Acc_Stat'); port_label('output', 76, 'BS_SS_Acc_Stat_SBSP'); port_label('output', 77, 'BS_SS_RqPerf_Stat'); port_label('output', 78, 'BS_SS_RqPerf_Stat_SBSP'); port_label('output', 79, 'ConfLatAccel_SBSP'); port_label('output', 80, 'ConfLgtAccel_SBSP'); port_label('output', 81, 'ConfYawRate_SBSP'); port_label('output', 82, 'EBS_BrkSw2_Rq'); port_label('output', 83, 'EBS_BrkSw2_Rq_SBSP'); port_label('output', 84, 'EngRetTrqMax_Rq'); port_label('output', 85, 'EngRetTrqMin_Rq'); port_label('output', 86, 'FoundBrk_Stat'); port_label('output', 87, 'FullBrkAllow_Stat_SBSP'); port_label('output', 88, 'GroCmbVehWeight_Cval'); port_label('output', 89, 'HillHolderAvl_Stat'); port_label('output', 90, 'NrTrlr_Stat_SBSP'); port_label('output', 91, 'PwrVehWeight_Cval'); port_label('output', 92, 'RoadCurv_Cval'); port_label('output', 93, 'ROP_BrkCtrlActv2_Stat'); port_label('output', 94, 'ROP_EngCtrlActv2_Stat'); port_label('output', 95, 'sAccel_X_Cval_SBSP'); port_label('output', 96, 'sAccel_Y_Cval_SBSP'); port_label('output', 97, 'sAddInfoVehSped_Cval_SBSP'); port_label('output', 98, 'sBrkPdlPosn3_Cval_SBSP'); port_label('output', 99, 'sBS_Brk_Cval_SBSP'); port_label('output', 100, 'sBS_CS_Acc_Stat_SBSP'); port_label('output', 101, 'sBS_CS_RqPerf2_Stat_SBSP'); port_label('output', 102, 'sBS_CS_RqPerf_Stat_SBSP'); port_label('output', 103, 'sBS_CSCPC_Acc_Stat_SBSP'); port_label('output', 104, 'sBS_HB_Acc_Stat_SBSP'); port_label('output', 105, 'sBS_HB_RqPerf_Stat_SBSP'); port_label('output', 106, 'sBS_HBCPC_Acc_Stat_SBSP'); port_label('output', 107, 'sBS_HBCPC_RqPerf_Stat_SBSP'); port_label('output', 108, 'sBS_SS_Acc_Stat_SBSP'); port_label('output', 109, 'sBS_SS_RqPerf_Stat_SBSP'); port_label('output', 110, 'sConfLatAccel_SBSP'); port_label('output', 111, 'sConfLgtAccel_SBSP'); port_label('output', 112, 'sConfYawRate_SBSP'); port_label('output', 113, 'sEBS_BrkSw2_Rq_SBSP'); port_label('output', 114, 'sFullBrkAllow_Stat_SBSP'); port_label('output', 115, 'SpdFtAxleLtWhl_Cval'); port_label('output', 116, 'SpdFtAxleLtWhl_Cval_SBSP'); port_label('output', 117, 'SpdFtAxleRtWhl_Cval'); port_label('output', 118, 'SpdFtAxleRtWhl_Cval_SBSP'); port_label('output', 119, 'SpdR_AxleLtWhl_Cval'); port_label('output', 120, 'SpdR_AxleLtWhl_Cval_SBSP'); port_label('output', 121, 'SpdR_AxleRtWhl_Cval'); port_label('output', 122, 'SpdR_AxleRtWhl_Cval_SBSP'); port_label('output', 123, 'SrcAdrBrkCtrlDev_Cval'); port_label('output', 124, 'SrcAdrBrkCtrlDev_Cval_SBSP'); port_label('output', 125, 'sSpdFtAxleLtWhl_Cval_SBSP'); port_label('output', 126, 'sSpdFtAxleRtWhl_Cval_SBSP'); port_label('output', 127, 'sSpdR_AxleLtWhl_Cval_SBSP'); port_label('output', 128, 'sSpdR_AxleRtWhl_Cval_SBSP'); port_label('output', 129, 'sSrcAdrBrkCtrlDev_Cval_SBSP'); port_label('output', 130, 'sStandstill_Dtct_Stat_SBSP'); port_label('output', 131, 'Standstill_Dtct_Stat_SBSP'); port_label('output', 132, 'sTrlrAbsOper_Stat'); port_label('output', 133, 'sTrlrEstm_Stat_SBSP'); port_label('output', 134, 'sVehSpd_Cval_SBSP'); port_label('output', 135, 'sXBR_AccelLim_Stat_SBSP'); port_label('output', 136, 'sXBR_ActCtrl_Stat_SBSP'); port_label('output', 137, 'sXBR_Sys_Stat_SBSP'); port_label('output', 138, 'sYawRateCorr_Cval_SBSP'); port_label('output', 139, 'TrctrAbsOper_Stat'); port_label('output', 140, 'TrlrAbsOper_Stat'); port_label('output', 141, 'TrlrEstm_Stat_SBSP'); port_label('output', 142, 'TyreCorrLtFA_Cval'); port_label('output', 143, 'TyreCorrLtRA_Cval'); port_label('output', 144, 'TyreCorrRtFA_Cval'); port_label('output', 145, 'TyreCorrRtRA_Cval'); port_label('output', 146, 'TyreRollCircumFA_Cval'); port_label('output', 147, 'TyreRollCircumRA_Cval'); port_label('output', 148, 'VehSpd_Cval_BS'); port_label('output', 149, 'VehSpd_Cval_SBSP'); port_label('output', 150, 'XBR_AccelLim_Stat_BS'); port_label('output', 151, 'XBR_AccelLim_Stat_SBSP'); port_label('output', 152, 'XBR_ActCtrl_Stat_SBSP'); port_label('output', 153, 'XBR_Sys_Stat_SBSP'); port_label('output', 154, 'YawRateCorr_Cval_SBSP'); port_label('output', 155, 'YC_BrkCtrlActv2_Stat'); port_label('output', 156, 'YC_EngCtrlActv2_Stat'); port_label('output', 157, 'ebs_ActlEmotTrq_Nm'); port_label('output', 158, 'ebs_ActlEngTrq_Nm'); port_label('output', 159, 'ebs_ActlRetTrq_Nm'); port_label('output', 160, 'ebs_i_Emot'); port_label('output', 161, 'ebs_i_Ret'); port_label('output', 162, 'ebs_kappa'); port_label('output', 163, 'ebs_SumBrakingForces_Trailer'); port_label('output', 164, 'ebs_SumBrakingForces_Vehicle'); port_label('output', 165, 'ebs_zReqBrake'); port_label('output', 166, 'ebs_zReqEB'); port_label('output', 167, 'ebs_zRet'); port_label('output', 168, 'ebs_zSlopeComp'); port_label('output', 169, 'ebs_zSoll_BWG');
  ebs_AdditionalAxle_left_pDmd : Outport
  ebs_AdditionalAxle_right_pDmd : Outport  Port=2
  ebs_ESCsens_y_acceleration : Outport  Port=3
  ebs_FrontAxle_left_pDmd : Outport  Port=4
  ebs_FrontAxle_right_pDmd : Outport  Port=5
  ebs_RearAxle_left_pDmd : Outport  Port=6
  ebs_RearAxle_right_pDmd : Outport  Port=7
  ebs_sBSP_stABSInValve_Addl_Left : Outport  Port=8
  ebs_sBSP_stABSInValve_Addl_Right : Outport  Port=9
  ebs_sBSP_stABSInValve_Front_Left : Outport  Port=10
  ebs_sBSP_stABSInValve_Front_Right : Outport  Port=11
  ebs_sBSP_stABSInValve_RCMax_Front : Outport  Port=12
  ebs_sBSP_stABSInValve_RCMax_Rear : Outport  Port=13
  ebs_sBSP_stABSInValve_Rear_Left : Outport  Port=14
  ebs_sBSP_stABSInValve_Rear_Right : Outport  Port=15
  ebs_sBSP_stABSOutValve_Addl_Left : Outport  Port=16
  ebs_sBSP_stABSOutValve_Addl_Right : Outport  Port=17
  ebs_sBSP_stABSOutValve_Front_Left : Outport  Port=18
  ebs_sBSP_stABSOutValve_Front_Right : Outport  Port=19
  ebs_sBSP_stABSOutValve_RCMax_Front : Outport  Port=20
  ebs_sBSP_stABSOutValve_RCMax_Rear : Outport  Port=21
  ebs_sBSP_stABSOutValve_Rear_Left : Outport  Port=22
  ebs_sBSP_stABSOutValve_Rear_Right : Outport  Port=23
  ebs_sBSP_stAPCVBuValve : Outport  Port=24
  ebs_sBSP_stAxmoBuValve : Outport  Port=25
  ebs_sBSP_stCMaxBuValve : Outport  Port=26
  ebs_TCV_pDmd : Outport  Port=27
  aAutoOpMd_Stat_SBSP : Outport  Port=28
  aBrkAirPressAA_Cval_SBSP : Outport  Port=29
  aBrkAirPressFA_Cval_SBSP : Outport  Port=30
  aBrkAirPressRA_Cval_SBSP : Outport  Port=31
  aBrkPdlPosn3_Cval_SBSP : Outport  Port=32
  aBrkTempFA_Cval_SBSP : Outport  Port=33
  aBrkTempIA_Cval_SBSP : Outport  Port=34
  aBrkTempRA_Cval_SBSP : Outport  Port=35
  ABS_Actv2_Stat : Outport  Port=36
  ABS_Actv_Stat : Outport  Port=37
  ABS_FullyOp_Stat : Outport  Port=38
  ABS_Trlr_Stat : Outport  Port=39
  Accel_X_Cval : Outport  Port=40
  Accel_X_Cval_SBSP : Outport  Port=41
  Accel_Y_Cval : Outport  Port=42
  Accel_Y_Cval_SBSP : Outport  Port=43
  AddInfoVehSped_Cval_SBSP : Outport  Port=44
  aGroCmbVehWeight_Cval_SBSP : Outport  Port=45
  aGroCmbVehWeightConf_SBSP : Outport  Port=46
  aStandstill_Dtct_Stat_SBSP : Outport  Port=47
  ATC_BrkCtrl_Stat : Outport  Port=48
  ATC_EngCtrl_Stat : Outport  Port=49
  ATC_InfoSgl_Stat : Outport  Port=50
  aTCV_Press_Cval_SBSP : Outport  Port=51
  aVehSpd_Cval_E2E_SBSP : Outport  Port=52
  aVehSpd_Cval_SBSP : Outport  Port=53
  BlockTend_Stat : Outport  Port=54
  BrkPdlPosn3_Cval : Outport  Port=55
  BrkPdlPosn3_Cval_SBSP : Outport  Port=56
  BrkPdlPosn_Cval : Outport  Port=57
  BS_Brk_Cval : Outport  Port=58
  BS_Brk_Cval_SBSP : Outport  Port=59
  BS_CS_Acc_Stat : Outport  Port=60
  BS_CS_Acc_Stat_SBSP : Outport  Port=61
  BS_CS_RqPerf2_Stat : Outport  Port=62
  BS_CS_RqPerf2_Stat_SBSP : Outport  Port=63
  BS_CS_RqPerf_Stat_SBSP : Outport  Port=64
  BS_CSCPC_Acc_Stat : Outport  Port=65
  BS_CSCPC_Acc_Stat_SBSP : Outport  Port=66
  BS_CSCPC_Intf_Stat : Outport  Port=67
  BS_CSCPC_RqPerf_Stat : Outport  Port=68
  BS_HB_Acc_Stat_SBSP : Outport  Port=69
  BS_HB_RqPerf_Stat : Outport  Port=70
  BS_HB_RqPerf_Stat_SBSP : Outport  Port=71
  BS_HBCPC_Acc_Stat_SBSP : Outport  Port=72
  BS_HBCPC_RqPerf_Stat_SBSP : Outport  Port=73
  BS_RoadIncln_Cval : Outport  Port=74
  BS_SS_Acc_Stat : Outport  Port=75
  BS_SS_Acc_Stat_SBSP : Outport  Port=76
  BS_SS_RqPerf_Stat : Outport  Port=77
  BS_SS_RqPerf_Stat_SBSP : Outport  Port=78
  ConfLatAccel_SBSP : Outport  Port=79
  ConfLgtAccel_SBSP : Outport  Port=80
  ConfYawRate_SBSP : Outport  Port=81
  EBS_BrkSw2_Rq : Outport  Port=82
  EBS_BrkSw2_Rq_SBSP : Outport  Port=83
  EngRetTrqMax_Rq : Outport  Port=84
  EngRetTrqMin_Rq : Outport  Port=85
  FoundBrk_Stat : Outport  Port=86
  FullBrkAllow_Stat_SBSP : Outport  Port=87
  GroCmbVehWeight_Cval : Outport  Port=88
  HillHolderAvl_Stat : Outport  Port=89
  NrTrlr_Stat_SBSP : Outport  Port=90
  PwrVehWeight_Cval : Outport  Port=91
  RoadCurv_Cval : Outport  Port=92
  ROP_BrkCtrlActv2_Stat : Outport  Port=93
  ROP_EngCtrlActv2_Stat : Outport  Port=94
  sAccel_X_Cval_SBSP : Outport  Port=95
  sAccel_Y_Cval_SBSP : Outport  Port=96
  sAddInfoVehSped_Cval_SBSP : Outport  Port=97
  sBrkPdlPosn3_Cval_SBSP : Outport  Port=98
  sBS_Brk_Cval_SBSP : Outport  Port=99
  sBS_CS_Acc_Stat_SBSP : Outport  Port=100
  sBS_CS_RqPerf2_Stat_SBSP : Outport  Port=101
  sBS_CS_RqPerf_Stat_SBSP : Outport  Port=102
  sBS_CSCPC_Acc_Stat_SBSP : Outport  Port=103
  sBS_HB_Acc_Stat_SBSP : Outport  Port=104
  sBS_HB_RqPerf_Stat_SBSP : Outport  Port=105
  sBS_HBCPC_Acc_Stat_SBSP : Outport  Port=106
  sBS_HBCPC_RqPerf_Stat_SBSP : Outport  Port=107
  sBS_SS_Acc_Stat_SBSP : Outport  Port=108
  sBS_SS_RqPerf_Stat_SBSP : Outport  Port=109
  sConfLatAccel_SBSP : Outport  Port=110
  sConfLgtAccel_SBSP : Outport  Port=111
  sConfYawRate_SBSP : Outport  Port=112
  sEBS_BrkSw2_Rq_SBSP : Outport  Port=113
  sFullBrkAllow_Stat_SBSP : Outport  Port=114
  SpdFtAxleLtWhl_Cval : Outport  Port=115
  SpdFtAxleLtWhl_Cval_SBSP : Outport  Port=116
  SpdFtAxleRtWhl_Cval : Outport  Port=117
  SpdFtAxleRtWhl_Cval_SBSP : Outport  Port=118
  SpdR_AxleLtWhl_Cval : Outport  Port=119
  SpdR_AxleLtWhl_Cval_SBSP : Outport  Port=120
  SpdR_AxleRtWhl_Cval : Outport  Port=121
  SpdR_AxleRtWhl_Cval_SBSP : Outport  Port=122
  SrcAdrBrkCtrlDev_Cval : Outport  Port=123
  SrcAdrBrkCtrlDev_Cval_SBSP : Outport  Port=124
  sSpdFtAxleLtWhl_Cval_SBSP : Outport  Port=125
  sSpdFtAxleRtWhl_Cval_SBSP : Outport  Port=126
  sSpdR_AxleLtWhl_Cval_SBSP : Outport  Port=127
  sSpdR_AxleRtWhl_Cval_SBSP : Outport  Port=128
  sSrcAdrBrkCtrlDev_Cval_SBSP : Outport  Port=129
  sStandstill_Dtct_Stat_SBSP : Outport  Port=130
  Standstill_Dtct_Stat_SBSP : Outport  Port=131
  sTrlrAbsOper_Stat : Outport  Port=132
  sTrlrEstm_Stat_SBSP : Outport  Port=133
  sVehSpd_Cval_SBSP : Outport  Port=134
  sXBR_AccelLim_Stat_SBSP : Outport  Port=135
  sXBR_ActCtrl_Stat_SBSP : Outport  Port=136
  sXBR_Sys_Stat_SBSP : Outport  Port=137
  sYawRateCorr_Cval_SBSP : Outport  Port=138
  TrctrAbsOper_Stat : Outport  Port=139
  TrlrAbsOper_Stat : Outport  Port=140
  TrlrEstm_Stat_SBSP : Outport  Port=141
  TyreCorrLtFA_Cval : Outport  Port=142
  TyreCorrLtRA_Cval : Outport  Port=143
  TyreCorrRtFA_Cval : Outport  Port=144
  TyreCorrRtRA_Cval : Outport  Port=145
  TyreRollCircumFA_Cval : Outport  Port=146
  TyreRollCircumRA_Cval : Outport  Port=147
  VehSpd_Cval_BS : Outport  Port=148
  VehSpd_Cval_SBSP : Outport  Port=149
  XBR_AccelLim_Stat_BS : Outport  Port=150
  XBR_AccelLim_Stat_SBSP : Outport  Port=151
  XBR_ActCtrl_Stat_SBSP : Outport  Port=152
  XBR_Sys_Stat_SBSP : Outport  Port=153
  YawRateCorr_Cval_SBSP : Outport  Port=154
  YC_BrkCtrlActv2_Stat : Outport  Port=155
  YC_EngCtrlActv2_Stat : Outport  Port=156
  ebs_ActlEmotTrq_Nm : Outport  Port=157
  ebs_ActlEngTrq_Nm : Outport  Port=158
  ebs_ActlRetTrq_Nm : Outport  Port=159
  ebs_i_Emot : Outport  Port=160
  ebs_i_Ret : Outport  Port=161
  ebs_kappa : Outport  Port=162
  ebs_SumBrakingForces_Trailer : Outport  Port=163
  ebs_SumBrakingForces_Vehicle : Outport  Port=164
  ebs_zReqBrake : Outport  Port=165
  ebs_zReqEB : Outport  Port=166
  ebs_zRet : Outport  Port=167
  ebs_zSlopeComp : Outport  Port=168
  ebs_zSoll_BWG : Outport  Port=169
  wires:
  ebs_rebuild_generic_std_sf/169 -> ebs_zSoll_BWG/1  "ebs_zSoll_BWG"
  ebs_rebuild_generic_std_sf/168 -> ebs_zSlopeComp/1  "ebs_zSlopeComp"
  ebs_rebuild_generic_std_sf/167 -> ebs_zRet/1  "ebs_zRet"
  ebs_rebuild_generic_std_sf/166 -> ebs_zReqEB/1  "ebs_zReqEB"
  ebs_rebuild_generic_std_sf/165 -> ebs_zReqBrake/1  "ebs_zReqBrake"
  ebs_rebuild_generic_std_sf/164 -> ebs_SumBrakingForces_Vehicle/1  "ebs_SumBrakingForces_Vehicle"
  ebs_rebuild_generic_std_sf/163 -> ebs_SumBrakingForces_Trailer/1  "ebs_SumBrakingForces_Trailer"
  ebs_rebuild_generic_std_sf/162 -> ebs_kappa/1  "ebs_kappa"
  ebs_rebuild_generic_std_sf/161 -> ebs_i_Ret/1  "ebs_i_Ret"
  ebs_rebuild_generic_std_sf/160 -> ebs_i_Emot/1  "ebs_i_Emot"
  ebs_rebuild_generic_std_sf/159 -> ebs_ActlRetTrq_Nm/1  "ebs_ActlRetTrq_Nm"
  ebs_rebuild_generic_std_sf/158 -> ebs_ActlEngTrq_Nm/1  "ebs_ActlEngTrq_Nm"
  ebs_rebuild_generic_std_sf/157 -> ebs_ActlEmotTrq_Nm/1  "ebs_ActlEmotTrq_Nm"
  ebs_rebuild_generic_std_sf/156 -> YC_EngCtrlActv2_Stat/1  "YC_EngCtrlActv2_Stat"
  ebs_rebuild_generic_std_sf/155 -> YC_BrkCtrlActv2_Stat/1  "YC_BrkCtrlActv2_Stat"
  ebs_rebuild_generic_std_sf/154 -> YawRateCorr_Cval_SBSP/1  "YawRateCorr_Cval_SBSP"
  ebs_rebuild_generic_std_sf/153 -> XBR_Sys_Stat_SBSP/1  "XBR_Sys_Stat_SBSP"
  ebs_rebuild_generic_std_sf/152 -> XBR_ActCtrl_Stat_SBSP/1  "XBR_ActCtrl_Stat_SBSP"
  ebs_rebuild_generic_std_sf/151 -> XBR_AccelLim_Stat_SBSP/1  "XBR_AccelLim_Stat_SBSP"
  ebs_rebuild_generic_std_sf/150 -> XBR_AccelLim_Stat_BS/1  "XBR_AccelLim_Stat_BS"
  ebs_rebuild_generic_std_sf/149 -> VehSpd_Cval_SBSP/1  "VehSpd_Cval_SBSP"
  ebs_rebuild_generic_std_sf/148 -> VehSpd_Cval_BS/1  "VehSpd_Cval_BS"
  ebs_rebuild_generic_std_sf/147 -> TyreRollCircumRA_Cval/1  "TyreRollCircumRA_Cval"
  ebs_rebuild_generic_std_sf/146 -> TyreRollCircumFA_Cval/1  "TyreRollCircumFA_Cval"
  ebs_rebuild_generic_std_sf/145 -> TyreCorrRtRA_Cval/1  "TyreCorrRtRA_Cval"
  ebs_rebuild_generic_std_sf/144 -> TyreCorrRtFA_Cval/1  "TyreCorrRtFA_Cval"
  ebs_rebuild_generic_std_sf/143 -> TyreCorrLtRA_Cval/1  "TyreCorrLtRA_Cval"
  ebs_rebuild_generic_std_sf/142 -> TyreCorrLtFA_Cval/1  "TyreCorrLtFA_Cval"
  ebs_rebuild_generic_std_sf/141 -> TrlrEstm_Stat_SBSP/1  "TrlrEstm_Stat_SBSP"
  ebs_rebuild_generic_std_sf/140 -> TrlrAbsOper_Stat/1  "TrlrAbsOper_Stat"
  ebs_rebuild_generic_std_sf/139 -> TrctrAbsOper_Stat/1  "TrctrAbsOper_Stat"
  ebs_rebuild_generic_std_sf/138 -> sYawRateCorr_Cval_SBSP/1  "sYawRateCorr_Cval_SBSP"
  ebs_rebuild_generic_std_sf/137 -> sXBR_Sys_Stat_SBSP/1  "sXBR_Sys_Stat_SBSP"
  ebs_rebuild_generic_std_sf/136 -> sXBR_ActCtrl_Stat_SBSP/1  "sXBR_ActCtrl_Stat_SBSP"
  ebs_rebuild_generic_std_sf/135 -> sXBR_AccelLim_Stat_SBSP/1  "sXBR_AccelLim_Stat_SBSP"
  ebs_rebuild_generic_std_sf/134 -> sVehSpd_Cval_SBSP/1  "sVehSpd_Cval_SBSP"
  ebs_rebuild_generic_std_sf/133 -> sTrlrEstm_Stat_SBSP/1  "sTrlrEstm_Stat_SBSP"
  ebs_rebuild_generic_std_sf/132 -> sTrlrAbsOper_Stat/1  "sTrlrAbsOper_Stat"
  ebs_rebuild_generic_std_sf/131 -> Standstill_Dtct_Stat_SBSP/1  "Standstill_Dtct_Stat_SBSP"
  ebs_rebuild_generic_std_sf/130 -> sStandstill_Dtct_Stat_SBSP/1  "sStandstill_Dtct_Stat_SBSP"
  ebs_rebuild_generic_std_sf/129 -> sSrcAdrBrkCtrlDev_Cval_SBSP/1  "sSrcAdrBrkCtrlDev_Cval_SBSP"
  ebs_rebuild_generic_std_sf/128 -> sSpdR_AxleRtWhl_Cval_SBSP/1  "sSpdR_AxleRtWhl_Cval_SBSP"
  ebs_rebuild_generic_std_sf/127 -> sSpdR_AxleLtWhl_Cval_SBSP/1  "sSpdR_AxleLtWhl_Cval_SBSP"
  ebs_rebuild_generic_std_sf/126 -> sSpdFtAxleRtWhl_Cval_SBSP/1  "sSpdFtAxleRtWhl_Cval_SBSP"
  ebs_rebuild_generic_std_sf/125 -> sSpdFtAxleLtWhl_Cval_SBSP/1  "sSpdFtAxleLtWhl_Cval_SBSP"
  ebs_rebuild_generic_std_sf/124 -> SrcAdrBrkCtrlDev_Cval_SBSP/1  "SrcAdrBrkCtrlDev_Cval_SBSP"
  ebs_rebuild_generic_std_sf/123 -> SrcAdrBrkCtrlDev_Cval/1  "SrcAdrBrkCtrlDev_Cval"
  ebs_rebuild_generic_std_sf/122 -> SpdR_AxleRtWhl_Cval_SBSP/1  "SpdR_AxleRtWhl_Cval_SBSP"
  ebs_rebuild_generic_std_sf/121 -> SpdR_AxleRtWhl_Cval/1  "SpdR_AxleRtWhl_Cval"
  ebs_rebuild_generic_std_sf/120 -> SpdR_AxleLtWhl_Cval_SBSP/1  "SpdR_AxleLtWhl_Cval_SBSP"
  ebs_rebuild_generic_std_sf/119 -> SpdR_AxleLtWhl_Cval/1  "SpdR_AxleLtWhl_Cval"
  ebs_rebuild_generic_std_sf/118 -> SpdFtAxleRtWhl_Cval_SBSP/1  "SpdFtAxleRtWhl_Cval_SBSP"
  ebs_rebuild_generic_std_sf/117 -> SpdFtAxleRtWhl_Cval/1  "SpdFtAxleRtWhl_Cval"
  ebs_rebuild_generic_std_sf/116 -> SpdFtAxleLtWhl_Cval_SBSP/1  "SpdFtAxleLtWhl_Cval_SBSP"
  ebs_rebuild_generic_std_sf/115 -> SpdFtAxleLtWhl_Cval/1  "SpdFtAxleLtWhl_Cval"
  ebs_rebuild_generic_std_sf/114 -> sFullBrkAllow_Stat_SBSP/1  "sFullBrkAllow_Stat_SBSP"
  ebs_rebuild_generic_std_sf/113 -> sEBS_BrkSw2_Rq_SBSP/1  "sEBS_BrkSw2_Rq_SBSP"
  ebs_rebuild_generic_std_sf/112 -> sConfYawRate_SBSP/1  "sConfYawRate_SBSP"
  ebs_rebuild_generic_std_sf/111 -> sConfLgtAccel_SBSP/1  "sConfLgtAccel_SBSP"
  ebs_rebuild_generic_std_sf/110 -> sConfLatAccel_SBSP/1  "sConfLatAccel_SBSP"
  ebs_rebuild_generic_std_sf/109 -> sBS_SS_RqPerf_Stat_SBSP/1  "sBS_SS_RqPerf_Stat_SBSP"
  ebs_rebuild_generic_std_sf/108 -> sBS_SS_Acc_Stat_SBSP/1  "sBS_SS_Acc_Stat_SBSP"
  ebs_rebuild_generic_std_sf/107 -> sBS_HBCPC_RqPerf_Stat_SBSP/1  "sBS_HBCPC_RqPerf_Stat_SBSP"
  ebs_rebuild_generic_std_sf/106 -> sBS_HBCPC_Acc_Stat_SBSP/1  "sBS_HBCPC_Acc_Stat_SBSP"
  ebs_rebuild_generic_std_sf/105 -> sBS_HB_RqPerf_Stat_SBSP/1  "sBS_HB_RqPerf_Stat_SBSP"
  ebs_rebuild_generic_std_sf/104 -> sBS_HB_Acc_Stat_SBSP/1  "sBS_HB_Acc_Stat_SBSP"
  ebs_rebuild_generic_std_sf/103 -> sBS_CSCPC_Acc_Stat_SBSP/1  "sBS_CSCPC_Acc_Stat_SBSP"
  ebs_rebuild_generic_std_sf/102 -> sBS_CS_RqPerf_Stat_SBSP/1  "sBS_CS_RqPerf_Stat_SBSP"
  ebs_rebuild_generic_std_sf/101 -> sBS_CS_RqPerf2_Stat_SBSP/1  "sBS_CS_RqPerf2_Stat_SBSP"
  ebs_rebuild_generic_std_sf/100 -> sBS_CS_Acc_Stat_SBSP/1  "sBS_CS_Acc_Stat_SBSP"
  ebs_rebuild_generic_std_sf/99 -> sBS_Brk_Cval_SBSP/1  "sBS_Brk_Cval_SBSP"
  ebs_rebuild_generic_std_sf/98 -> sBrkPdlPosn3_Cval_SBSP/1  "sBrkPdlPosn3_Cval_SBSP"
  ebs_rebuild_generic_std_sf/97 -> sAddInfoVehSped_Cval_SBSP/1  "sAddInfoVehSped_Cval_SBSP"
  ebs_rebuild_generic_std_sf/96 -> sAccel_Y_Cval_SBSP/1  "sAccel_Y_Cval_SBSP"
  ebs_rebuild_generic_std_sf/95 -> sAccel_X_Cval_SBSP/1  "sAccel_X_Cval_SBSP"
  ebs_rebuild_generic_std_sf/94 -> ROP_EngCtrlActv2_Stat/1  "ROP_EngCtrlActv2_Stat"
  ebs_rebuild_generic_std_sf/93 -> ROP_BrkCtrlActv2_Stat/1  "ROP_BrkCtrlActv2_Stat"
  ebs_rebuild_generic_std_sf/92 -> RoadCurv_Cval/1  "RoadCurv_Cval"
  ebs_rebuild_generic_std_sf/91 -> PwrVehWeight_Cval/1  "PwrVehWeight_Cval"
  ebs_rebuild_generic_std_sf/90 -> NrTrlr_Stat_SBSP/1  "NrTrlr_Stat_SBSP"
  ebs_rebuild_generic_std_sf/89 -> HillHolderAvl_Stat/1  "HillHolderAvl_Stat"
  ebs_rebuild_generic_std_sf/88 -> GroCmbVehWeight_Cval/1  "GroCmbVehWeight_Cval"
  ebs_rebuild_generic_std_sf/87 -> FullBrkAllow_Stat_SBSP/1  "FullBrkAllow_Stat_SBSP"
  ebs_rebuild_generic_std_sf/86 -> FoundBrk_Stat/1  "FoundBrk_Stat"
  ebs_rebuild_generic_std_sf/85 -> EngRetTrqMin_Rq/1  "EngRetTrqMin_Rq"
  ebs_rebuild_generic_std_sf/84 -> EngRetTrqMax_Rq/1  "EngRetTrqMax_Rq"
  ebs_rebuild_generic_std_sf/83 -> EBS_BrkSw2_Rq_SBSP/1  "EBS_BrkSw2_Rq_SBSP"
  ebs_rebuild_generic_std_sf/82 -> EBS_BrkSw2_Rq/1  "EBS_BrkSw2_Rq"
  ebs_rebuild_generic_std_sf/81 -> ConfYawRate_SBSP/1  "ConfYawRate_SBSP"
  ebs_rebuild_generic_std_sf/80 -> ConfLgtAccel_SBSP/1  "ConfLgtAccel_SBSP"
  ebs_rebuild_generic_std_sf/79 -> ConfLatAccel_SBSP/1  "ConfLatAccel_SBSP"
  ebs_rebuild_generic_std_sf/78 -> BS_SS_RqPerf_Stat_SBSP/1  "BS_SS_RqPerf_Stat_SBSP"
  ebs_rebuild_generic_std_sf/77 -> BS_SS_RqPerf_Stat/1  "BS_SS_RqPerf_Stat"
  ebs_rebuild_generic_std_sf/76 -> BS_SS_Acc_Stat_SBSP/1  "BS_SS_Acc_Stat_SBSP"
  ebs_rebuild_generic_std_sf/75 -> BS_SS_Acc_Stat/1  "BS_SS_Acc_Stat"
  ebs_rebuild_generic_std_sf/74 -> BS_RoadIncln_Cval/1  "BS_RoadIncln_Cval"
  ebs_rebuild_generic_std_sf/73 -> BS_HBCPC_RqPerf_Stat_SBSP/1  "BS_HBCPC_RqPerf_Stat_SBSP"
  ebs_rebuild_generic_std_sf/72 -> BS_HBCPC_Acc_Stat_SBSP/1  "BS_HBCPC_Acc_Stat_SBSP"
  ebs_rebuild_generic_std_sf/71 -> BS_HB_RqPerf_Stat_SBSP/1  "BS_HB_RqPerf_Stat_SBSP"
  ebs_rebuild_generic_std_sf/70 -> BS_HB_RqPerf_Stat/1  "BS_HB_RqPerf_Stat"
  ebs_rebuild_generic_std_sf/69 -> BS_HB_Acc_Stat_SBSP/1  "BS_HB_Acc_Stat_SBSP"
  ebs_rebuild_generic_std_sf/68 -> BS_CSCPC_RqPerf_Stat/1  "BS_CSCPC_RqPerf_Stat"
  ebs_rebuild_generic_std_sf/67 -> BS_CSCPC_Intf_Stat/1  "BS_CSCPC_Intf_Stat"
  ebs_rebuild_generic_std_sf/66 -> BS_CSCPC_Acc_Stat_SBSP/1  "BS_CSCPC_Acc_Stat_SBSP"
  ebs_rebuild_generic_std_sf/65 -> BS_CSCPC_Acc_Stat/1  "BS_CSCPC_Acc_Stat"
  ebs_rebuild_generic_std_sf/64 -> BS_CS_RqPerf_Stat_SBSP/1  "BS_CS_RqPerf_Stat_SBSP"
  ebs_rebuild_generic_std_sf/63 -> BS_CS_RqPerf2_Stat_SBSP/1  "BS_CS_RqPerf2_Stat_SBSP"
  ebs_rebuild_generic_std_sf/62 -> BS_CS_RqPerf2_Stat/1  "BS_CS_RqPerf2_Stat"
  ebs_rebuild_generic_std_sf/61 -> BS_CS_Acc_Stat_SBSP/1  "BS_CS_Acc_Stat_SBSP"
  ebs_rebuild_generic_std_sf/60 -> BS_CS_Acc_Stat/1  "BS_CS_Acc_Stat"
  ebs_rebuild_generic_std_sf/59 -> BS_Brk_Cval_SBSP/1  "BS_Brk_Cval_SBSP"
  ebs_rebuild_generic_std_sf/58 -> BS_Brk_Cval/1  "BS_Brk_Cval"
  ebs_rebuild_generic_std_sf/57 -> BrkPdlPosn_Cval/1  "BrkPdlPosn_Cval"
  ebs_rebuild_generic_std_sf/56 -> BrkPdlPosn3_Cval_SBSP/1  "BrkPdlPosn3_Cval_SBSP"
  ebs_rebuild_generic_std_sf/55 -> BrkPdlPosn3_Cval/1  "BrkPdlPosn3_Cval"
  ebs_rebuild_generic_std_sf/54 -> BlockTend_Stat/1  "BlockTend_Stat"
  ebs_rebuild_generic_std_sf/53 -> aVehSpd_Cval_SBSP/1  "aVehSpd_Cval_SBSP"
  ebs_rebuild_generic_std_sf/52 -> aVehSpd_Cval_E2E_SBSP/1  "aVehSpd_Cval_E2E_SBSP"
  ebs_rebuild_generic_std_sf/51 -> aTCV_Press_Cval_SBSP/1  "aTCV_Press_Cval_SBSP"
  ebs_rebuild_generic_std_sf/50 -> ATC_InfoSgl_Stat/1  "ATC_InfoSgl_Stat"
  ebs_rebuild_generic_std_sf/49 -> ATC_EngCtrl_Stat/1  "ATC_EngCtrl_Stat"
  ebs_rebuild_generic_std_sf/48 -> ATC_BrkCtrl_Stat/1  "ATC_BrkCtrl_Stat"
  ebs_rebuild_generic_std_sf/47 -> aStandstill_Dtct_Stat_SBSP/1  "aStandstill_Dtct_Stat_SBSP"
  ebs_rebuild_generic_std_sf/46 -> aGroCmbVehWeightConf_SBSP/1  "aGroCmbVehWeightConf_SBSP"
  ebs_rebuild_generic_std_sf/45 -> aGroCmbVehWeight_Cval_SBSP/1  "aGroCmbVehWeight_Cval_SBSP"
  ebs_rebuild_generic_std_sf/44 -> AddInfoVehSped_Cval_SBSP/1  "AddInfoVehSped_Cval_SBSP"
  ebs_rebuild_generic_std_sf/43 -> Accel_Y_Cval_SBSP/1  "Accel_Y_Cval_SBSP"
  ebs_rebuild_generic_std_sf/42 -> Accel_Y_Cval/1  "Accel_Y_Cval"
  ebs_rebuild_generic_std_sf/41 -> Accel_X_Cval_SBSP/1  "Accel_X_Cval_SBSP"
  ebs_rebuild_generic_std_sf/40 -> Accel_X_Cval/1  "Accel_X_Cval"
  ebs_rebuild_generic_std_sf/39 -> ABS_Trlr_Stat/1  "ABS_Trlr_Stat"
  ebs_rebuild_generic_std_sf/38 -> ABS_FullyOp_Stat/1  "ABS_FullyOp_Stat"
  ebs_rebuild_generic_std_sf/37 -> ABS_Actv_Stat/1  "ABS_Actv_Stat"
  ebs_rebuild_generic_std_sf/36 -> ABS_Actv2_Stat/1  "ABS_Actv2_Stat"
  ebs_rebuild_generic_std_sf/35 -> aBrkTempRA_Cval_SBSP/1  "aBrkTempRA_Cval_SBSP"
  ebs_rebuild_generic_std_sf/34 -> aBrkTempIA_Cval_SBSP/1  "aBrkTempIA_Cval_SBSP"
  ebs_rebuild_generic_std_sf/33 -> aBrkTempFA_Cval_SBSP/1  "aBrkTempFA_Cval_SBSP"
  ebs_rebuild_generic_std_sf/32 -> aBrkPdlPosn3_Cval_SBSP/1  "aBrkPdlPosn3_Cval_SBSP"
  ebs_rebuild_generic_std_sf/31 -> aBrkAirPressRA_Cval_SBSP/1  "aBrkAirPressRA_Cval_SBSP"
  ebs_rebuild_generic_std_sf/30 -> aBrkAirPressFA_Cval_SBSP/1  "aBrkAirPressFA_Cval_SBSP"
  ebs_rebuild_generic_std_sf/29 -> aBrkAirPressAA_Cval_SBSP/1  "aBrkAirPressAA_Cval_SBSP"
  ebs_rebuild_generic_std_sf/28 -> aAutoOpMd_Stat_SBSP/1  "aAutoOpMd_Stat_SBSP"
  ebs_rebuild_generic_std_sf/27 -> ebs_TCV_pDmd/1  "ebs_TCV_pDmd"
  ebs_rebuild_generic_std_sf/26 -> ebs_sBSP_stCMaxBuValve/1  "ebs_sBSP_stCMaxBuValve"
  ebs_rebuild_generic_std_sf/25 -> ebs_sBSP_stAxmoBuValve/1  "ebs_sBSP_stAxmoBuValve"
  ebs_rebuild_generic_std_sf/24 -> ebs_sBSP_stAPCVBuValve/1  "ebs_sBSP_stAPCVBuValve"
  ebs_rebuild_generic_std_sf/23 -> ebs_sBSP_stABSOutValve_Rear_Right/1  "ebs_sBSP_stABSOutValve_Rear_Right"
  ebs_rebuild_generic_std_sf/22 -> ebs_sBSP_stABSOutValve_Rear_Left/1  "ebs_sBSP_stABSOutValve_Rear_Left"
  ebs_rebuild_generic_std_sf/21 -> ebs_sBSP_stABSOutValve_RCMax_Rear/1  "ebs_sBSP_stABSOutValve_RCMax_Rear"
  ebs_rebuild_generic_std_sf/20 -> ebs_sBSP_stABSOutValve_RCMax_Front/1  "ebs_sBSP_stABSOutValve_RCMax_Front"
  ebs_rebuild_generic_std_sf/19 -> ebs_sBSP_stABSOutValve_Front_Right/1  "ebs_sBSP_stABSOutValve_Front_Right"
  ebs_rebuild_generic_std_sf/18 -> ebs_sBSP_stABSOutValve_Front_Left/1  "ebs_sBSP_stABSOutValve_Front_Left"
  ebs_rebuild_generic_std_sf/17 -> ebs_sBSP_stABSOutValve_Addl_Right/1  "ebs_sBSP_stABSOutValve_Addl_Right"
  ebs_rebuild_generic_std_sf/16 -> ebs_sBSP_stABSOutValve_Addl_Left/1  "ebs_sBSP_stABSOutValve_Addl_Left"
  ebs_rebuild_generic_std_sf/15 -> ebs_sBSP_stABSInValve_Rear_Right/1  "ebs_sBSP_stABSInValve_Rear_Right"
  ebs_rebuild_generic_std_sf/14 -> ebs_sBSP_stABSInValve_Rear_Left/1  "ebs_sBSP_stABSInValve_Rear_Left"
  ebs_rebuild_generic_std_sf/13 -> ebs_sBSP_stABSInValve_RCMax_Rear/1  "ebs_sBSP_stABSInValve_RCMax_Rear"
  ebs_rebuild_generic_std_sf/12 -> ebs_sBSP_stABSInValve_RCMax_Front/1  "ebs_sBSP_stABSInValve_RCMax_Front"
  ebs_rebuild_generic_std_sf/11 -> ebs_sBSP_stABSInValve_Front_Right/1  "ebs_sBSP_stABSInValve_Front_Right"
  ebs_rebuild_generic_std_sf/10 -> ebs_sBSP_stABSInValve_Front_Left/1  "ebs_sBSP_stABSInValve_Front_Left"
  ebs_rebuild_generic_std_sf/9 -> ebs_sBSP_stABSInValve_Addl_Right/1  "ebs_sBSP_stABSInValve_Addl_Right"
  ebs_rebuild_generic_std_sf/8 -> ebs_sBSP_stABSInValve_Addl_Left/1  "ebs_sBSP_stABSInValve_Addl_Left"
  ebs_rebuild_generic_std_sf/7 -> ebs_RearAxle_right_pDmd/1  "ebs_RearAxle_right_pDmd"
  ebs_rebuild_generic_std_sf/6 -> ebs_RearAxle_left_pDmd/1  "ebs_RearAxle_left_pDmd"
  ebs_rebuild_generic_std_sf/5 -> ebs_FrontAxle_right_pDmd/1  "ebs_FrontAxle_right_pDmd"
  ebs_rebuild_generic_std_sf/4 -> ebs_FrontAxle_left_pDmd/1  "ebs_FrontAxle_left_pDmd"
  ebs_rebuild_generic_std_sf/3 -> ebs_ESCsens_y_acceleration/1  "ebs_ESCsens_y_acceleration"
  ebs_rebuild_generic_std_sf/2 -> ebs_AdditionalAxle_right_pDmd/1  "ebs_AdditionalAxle_right_pDmd"
  ebs_rebuild_generic_std_sf/1 -> ebs_AdditionalAxle_left_pDmd/1  "ebs_AdditionalAxle_left_pDmd"
  pne_brk_TrailerAxle3_torque_sns/1 -> ebs_rebuild_generic_std_sf/97  "pne_brk_TrailerAxle3_torque_sns"
  pne_brk_TrailerAxle3_BrakingForce_at8p5bar/1 -> ebs_rebuild_generic_std_sf/96  "pne_brk_TrailerAxle3_BrakingForce_at8p5bar"
  pne_brk_TrailerAxle2_torque_sns/1 -> ebs_rebuild_generic_std_sf/95  "pne_brk_TrailerAxle2_torque_sns"
  pne_brk_TrailerAxle2_BrakingForce_at8p5bar/1 -> ebs_rebuild_generic_std_sf/94  "pne_brk_TrailerAxle2_BrakingForce_at8p5bar"
  pne_brk_TrailerAxle1_torque_sns/1 -> ebs_rebuild_generic_std_sf/93  "pne_brk_TrailerAxle1_torque_sns"
  pne_brk_TrailerAxle1_BrakingForce_at8p5bar/1 -> ebs_rebuild_generic_std_sf/92  "pne_brk_TrailerAxle1_BrakingForce_at8p5bar"
  pne_brk_Trailer02Axle6_torque_sns/1 -> ebs_rebuild_generic_std_sf/91  "pne_brk_Trailer02Axle6_torque_sns"
  pne_brk_Trailer02Axle6_BrakingForce_at8p5bar/1 -> ebs_rebuild_generic_std_sf/90  "pne_brk_Trailer02Axle6_BrakingForce_at8p5bar"
  pne_brk_Trailer02Axle5_torque_sns/1 -> ebs_rebuild_generic_std_sf/89  "pne_brk_Trailer02Axle5_torque_sns"
  pne_brk_Trailer02Axle5_BrakingForce_at8p5bar/1 -> ebs_rebuild_generic_std_sf/88  "pne_brk_Trailer02Axle5_BrakingForce_at8p5bar"
  pne_brk_Trailer02Axle4_torque_sns/1 -> ebs_rebuild_generic_std_sf/87  "pne_brk_Trailer02Axle4_torque_sns"
  pne_brk_Trailer02Axle4_BrakingForce_at8p5bar/1 -> ebs_rebuild_generic_std_sf/86  "pne_brk_Trailer02Axle4_BrakingForce_at8p5bar"
  pne_brk_Trailer02Axle3_torque_sns/1 -> ebs_rebuild_generic_std_sf/85  "pne_brk_Trailer02Axle3_torque_sns"
  pne_brk_Trailer02Axle3_BrakingForce_at8p5bar/1 -> ebs_rebuild_generic_std_sf/84  "pne_brk_Trailer02Axle3_BrakingForce_at8p5bar"
  pne_brk_Trailer02Axle2_torque_sns/1 -> ebs_rebuild_generic_std_sf/83  "pne_brk_Trailer02Axle2_torque_sns"
  pne_brk_Trailer02Axle2_BrakingForce_at8p5bar/1 -> ebs_rebuild_generic_std_sf/82  "pne_brk_Trailer02Axle2_BrakingForce_at8p5bar"
  pne_brk_Trailer02Axle1_torque_sns/1 -> ebs_rebuild_generic_std_sf/81  "pne_brk_Trailer02Axle1_torque_sns"
  pne_brk_Trailer02Axle1_BrakingForce_at8p5bar/1 -> ebs_rebuild_generic_std_sf/80  "pne_brk_Trailer02Axle1_BrakingForce_at8p5bar"
  pne_brk_TCV_pAct/1 -> ebs_rebuild_generic_std_sf/79  "pne_brk_TCV_pAct"
  pne_brk_rotVel_rr/1 -> ebs_rebuild_generic_std_sf/78  "pne_brk_rotVel_rr"
  pne_brk_rotVel_rl/1 -> ebs_rebuild_generic_std_sf/77  "pne_brk_rotVel_rl"
  pne_brk_rotVel_fr/1 -> ebs_rebuild_generic_std_sf/76  "pne_brk_rotVel_fr"
  pne_brk_rotVel_fl/1 -> ebs_rebuild_generic_std_sf/75  "pne_brk_rotVel_fl"
  pne_brk_rotVel_ar/1 -> ebs_rebuild_generic_std_sf/74  "pne_brk_rotVel_ar"
  pne_brk_rotVel_al/1 -> ebs_rebuild_generic_std_sf/73  "pne_brk_rotVel_al"
  pne_brk_RearAxle_right_pAct/1 -> ebs_rebuild_generic_std_sf/72  "pne_brk_RearAxle_right_pAct"
  pne_brk_RearAxle_left_pAct/1 -> ebs_rebuild_generic_std_sf/71  "pne_brk_RearAxle_left_pAct"
  pne_brk_FrontAxle_pAct/1 -> ebs_rebuild_generic_std_sf/70  "pne_brk_FrontAxle_pAct"
  pne_brk_Axle4_torque_sns/1 -> ebs_rebuild_generic_std_sf/69  "pne_brk_Axle4_torque_sns"
  pne_brk_Axle4_right_Tinterior/1 -> ebs_rebuild_generic_std_sf/68  "pne_brk_Axle4_right_Tinterior"
  pne_brk_Axle4_left_Tinterior/1 -> ebs_rebuild_generic_std_sf/67  "pne_brk_Axle4_left_Tinterior"
  pne_brk_Axle4_BrakingForce_at8p5bar/1 -> ebs_rebuild_generic_std_sf/66  "pne_brk_Axle4_BrakingForce_at8p5bar"
  pne_brk_Axle3_torque_sns/1 -> ebs_rebuild_generic_std_sf/65  "pne_brk_Axle3_torque_sns"
  pne_brk_Axle3_right_Tinterior/1 -> ebs_rebuild_generic_std_sf/64  "pne_brk_Axle3_right_Tinterior"
  pne_brk_Axle3_left_Tinterior/1 -> ebs_rebuild_generic_std_sf/63  "pne_brk_Axle3_left_Tinterior"
  pne_brk_Axle3_BrakingForce_at8p5bar/1 -> ebs_rebuild_generic_std_sf/62  "pne_brk_Axle3_BrakingForce_at8p5bar"
  pne_brk_Axle2_torque_sns/1 -> ebs_rebuild_generic_std_sf/61  "pne_brk_Axle2_torque_sns"
  pne_brk_Axle2_right_Tinterior/1 -> ebs_rebuild_generic_std_sf/60  "pne_brk_Axle2_right_Tinterior"
  pne_brk_Axle2_left_Tinterior/1 -> ebs_rebuild_generic_std_sf/59  "pne_brk_Axle2_left_Tinterior"
  pne_brk_Axle2_BrakingForce_at8p5bar/1 -> ebs_rebuild_generic_std_sf/58  "pne_brk_Axle2_BrakingForce_at8p5bar"
  pne_brk_Axle1_torque_sns/1 -> ebs_rebuild_generic_std_sf/57  "pne_brk_Axle1_torque_sns"
  pne_brk_Axle1_right_Tinterior/1 -> ebs_rebuild_generic_std_sf/56  "pne_brk_Axle1_right_Tinterior"
  pne_brk_Axle1_left_Tinterior/1 -> ebs_rebuild_generic_std_sf/55  "pne_brk_Axle1_left_Tinterior"
  pne_brk_Axle1_BrakingForce_at8p5bar/1 -> ebs_rebuild_generic_std_sf/54  "pne_brk_Axle1_BrakingForce_at8p5bar"
  pne_brk_AdditionalAxle_right_pAct/1 -> ebs_rebuild_generic_std_sf/53  "pne_brk_AdditionalAxle_right_pAct"
  pne_brk_AdditionalAxle_left_pAct/1 -> ebs_rebuild_generic_std_sf/52  "pne_brk_AdditionalAxle_left_pAct"
  mec_veh_transVel/1 -> ebs_rebuild_generic_std_sf/51  "mec_veh_transVel"
  mec_veh_TrailerAxleLoad3/1 -> ebs_rebuild_generic_std_sf/50  "mec_veh_TrailerAxleLoad3"
  mec_veh_TrailerAxleLoad2/1 -> ebs_rebuild_generic_std_sf/49  "mec_veh_TrailerAxleLoad2"
  mec_veh_TrailerAxleLoad1/1 -> ebs_rebuild_generic_std_sf/48  "mec_veh_TrailerAxleLoad1"
  mec_veh_Trailer02AxleLoad6/1 -> ebs_rebuild_generic_std_sf/47  "mec_veh_Trailer02AxleLoad6"
  mec_veh_Trailer02AxleLoad5/1 -> ebs_rebuild_generic_std_sf/46  "mec_veh_Trailer02AxleLoad5"
  mec_veh_Trailer02AxleLoad4/1 -> ebs_rebuild_generic_std_sf/45  "mec_veh_Trailer02AxleLoad4"
  mec_veh_Trailer02AxleLoad3/1 -> ebs_rebuild_generic_std_sf/44  "mec_veh_Trailer02AxleLoad3"
  mec_veh_Trailer02AxleLoad2/1 -> ebs_rebuild_generic_std_sf/43  "mec_veh_Trailer02AxleLoad2"
  mec_veh_Trailer02AxleLoad1/1 -> ebs_rebuild_generic_std_sf/42  "mec_veh_Trailer02AxleLoad1"
  mec_veh_AxleLoad4/1 -> ebs_rebuild_generic_std_sf/41  "mec_veh_AxleLoad4"
  mec_veh_AxleLoad3/1 -> ebs_rebuild_generic_std_sf/40  "mec_veh_AxleLoad3"
  mec_veh_AxleLoad2/1 -> ebs_rebuild_generic_std_sf/39  "mec_veh_AxleLoad2"
  mec_veh_AxleLoad1/1 -> ebs_rebuild_generic_std_sf/38  "mec_veh_AxleLoad1"
  mec3d_ESCsens_y_acceleration/1 -> ebs_rebuild_generic_std_sf/37  "mec3d_ESCsens_y_acceleration"
  mec3d_ESCsens_gamma_rate/1 -> ebs_rebuild_generic_std_sf/36  "mec3d_ESCsens_gamma_rate"
  drv_PkBrk/1 -> ebs_rebuild_generic_std_sf/35  "drv_PkBrk"
  drv_BrkPdl_pos/1 -> ebs_rebuild_generic_std_sf/34  "drv_BrkPdl_pos"
  XBR_Prio_Stat_VRDU/1 -> ebs_rebuild_generic_std_sf/33  "XBR_Prio_Stat_VRDU"
  XBR_Prio_Stat_CPC5ce/1 -> ebs_rebuild_generic_std_sf/32  "XBR_Prio_Stat_CPC5ce"
  XBR_EBI_Stat_VRDU/1 -> ebs_rebuild_generic_std_sf/31  "XBR_EBI_Stat_VRDU"
  XBR_CtrlMode_Stat_VRDU/1 -> ebs_rebuild_generic_std_sf/30  "XBR_CtrlMode_Stat_VRDU"
  XBR_CtrlMode_Stat_CPC5ce/1 -> ebs_rebuild_generic_std_sf/29  "XBR_CtrlMode_Stat_CPC5ce"
  VehSpd1_Cval_Trlr/1 -> ebs_rebuild_generic_std_sf/28  "VehSpd1_Cval_Trlr"
  TxInShaftSpd_Cval_CPC/1 -> ebs_rebuild_generic_std_sf/27  "TxInShaftSpd_Cval_CPC"
  TrqConv_Cval_PT/1 -> ebs_rebuild_generic_std_sf/26  "TrqConv_Cval_PT"
  RetRefTrq_Cval/1 -> ebs_rebuild_generic_std_sf/25  "RetRefTrq_Cval"
  RetPctTrqActl2_Cval_CPC3/1 -> ebs_rebuild_generic_std_sf/24  "RetPctTrqActl2_Cval_CPC3"
  PkBrk_Rq_VRDU/1 -> ebs_rebuild_generic_std_sf/23  "PkBrk_Rq_VRDU"
  NomFrictEngPctTrq_Cval/1 -> ebs_rebuild_generic_std_sf/22  "NomFrictEngPctTrq_Cval"
  MinAvlEmotTrq_Cval_CPC/1 -> ebs_rebuild_generic_std_sf/21  "MinAvlEmotTrq_Cval_CPC"
  HB_Rq_Stat_VRDU/1 -> ebs_rebuild_generic_std_sf/20  "HB_Rq_Stat_VRDU"
  HB_Rq_Stat_CPC/1 -> ebs_rebuild_generic_std_sf/19  "HB_Rq_Stat_CPC"
  ExtBrkStat_Rq_VRDU/1 -> ebs_rebuild_generic_std_sf/18  "ExtBrkStat_Rq_VRDU"
  ExtBrkStat_Rq_CPC/1 -> ebs_rebuild_generic_std_sf/17  "ExtBrkStat_Rq_CPC"
  ExtAccel_Rq_VRDU3/1 -> ebs_rebuild_generic_std_sf/16  "ExtAccel_Rq_VRDU3"
  ExtAccel_Rq_VRDU/1 -> ebs_rebuild_generic_std_sf/15  "ExtAccel_Rq_VRDU"
  ExtAccel_Rq_CPC5ce/1 -> ebs_rebuild_generic_std_sf/14  "ExtAccel_Rq_CPC5ce"
  ExtAccel_Rq_CPC/1 -> ebs_rebuild_generic_std_sf/13  "ExtAccel_Rq_CPC"
  EngRPM_Cval_CPC3/1 -> ebs_rebuild_generic_std_sf/12  "EngRPM_Cval_CPC3"
  EngRefTrq_Cval/1 -> ebs_rebuild_generic_std_sf/11  "EngRefTrq_Cval"
  EngPctTrqActl_Cval/1 -> ebs_rebuild_generic_std_sf/10  "EngPctTrqActl_Cval"
  EdrvRefTrq_Cval/1 -> ebs_rebuild_generic_std_sf/9  "EdrvRefTrq_Cval"
  Clutch_Stat_CPC/1 -> ebs_rebuild_generic_std_sf/8  "Clutch_Stat_CPC"
  BrkPress_Rq/1 -> ebs_rebuild_generic_std_sf/7  "BrkPress_Rq"
  aSbspVehBrkForce_Cmd_SDS/1 -> ebs_rebuild_generic_std_sf/6  "aSbspVehBrkForce_Cmd_SDS"
  ActlMaxAvlRetPctTrq_Cval_CPC3/1 -> ebs_rebuild_generic_std_sf/5  "ActlMaxAvlRetPctTrq_Cval_CPC3"
  ActlEngPctTrq_Cval/1 -> ebs_rebuild_generic_std_sf/4  "ActlEngPctTrq_Cval"
  ActlEmotTrq_Cval/1 -> ebs_rebuild_generic_std_sf/3  "ActlEmotTrq_Cval"
  env_road_slope_pct/1 -> ebs_rebuild_generic_std_sf/2  "env_road_slope_pct"
  env_curv_pm/1 -> ebs_rebuild_generic_std_sf/1  "env_curv_pm"
